simulink model "model"  (R2016a)
(part 5 of 5)

  _CN_100861711_400000_CN_90547679_400000/RConn1 -- T_100861711_400000_Keadby_400kV_Substation/LConn1 -- _CN_100861711_400000_CN_257311344_400000/LConn1 -- _CN_100861711_400000_CN_160279525_400000/LConn1 -- _CN_100861711_400000_CN_204918278_400000/LConn1 -- _CN_100861711_400000_CN_205132633_400000/LConn1 -- _CN_100861711_400000_CN_33917128_400000/LConn1 -- _CN_100861711_400000_CN_58736682_400000/LConn1 -- _CN_100861711_400000_CN_324880597_400000/LConn1 -- _CN_100861711_400000_CN_159736514_400000/LConn1 -- _CN_100861711_400000_CN_34383063_400000/LConn1
  _CN_100861711_400000_CN_90547679_400000/RConn2 -- T_100861711_400000_Keadby_400kV_Substation/LConn2 -- _CN_100861711_400000_CN_257311344_400000/LConn2 -- _CN_100861711_400000_CN_160279525_400000/LConn2 -- _CN_100861711_400000_CN_204918278_400000/LConn2 -- _CN_100861711_400000_CN_205132633_400000/LConn2 -- _CN_100861711_400000_CN_33917128_400000/LConn2 -- _CN_100861711_400000_CN_58736682_400000/LConn2 -- _CN_100861711_400000_CN_324880597_400000/LConn2 -- _CN_100861711_400000_CN_159736514_400000/LConn2 -- _CN_100861711_400000_CN_34383063_400000/LConn2
  _CN_100861711_400000_CN_90547679_400000/RConn3 -- T_100861711_400000_Keadby_400kV_Substation/LConn3 -- _CN_100861711_400000_CN_257311344_400000/LConn3 -- _CN_100861711_400000_CN_160279525_400000/LConn3 -- _CN_100861711_400000_CN_204918278_400000/LConn3 -- _CN_100861711_400000_CN_205132633_400000/LConn3 -- _CN_100861711_400000_CN_33917128_400000/LConn3 -- _CN_100861711_400000_CN_58736682_400000/LConn3 -- _CN_100861711_400000_CN_324880597_400000/LConn3 -- bus109/LConn1 -- _CN_100861711_400000_CN_159736514_400000/LConn3 -- _CN_100861711_400000_CN_34383063_400000/LConn3
  T_159736514_400000;275000_Brinsworth_Switching_Station/LConn1 -- _CN_100861711_400000_CN_159736514_400000/RConn1
  T_159736514_400000;275000_Brinsworth_Switching_Station/LConn2 -- _CN_100861711_400000_CN_159736514_400000/RConn2
  _CN_100861711_400000_CN_159736514_400000/RConn3 -- T_159736514_400000;275000_Brinsworth_Switching_Station/LConn3 -- bus110/LConn1
  _CN_100861711_400000_CN_34383063_400000/RConn1 -- G_34383063_Drax_power_station/RConn1 -- _CN_160580052_400000_CN_34383063_400000/LConn1 -- _CN_25629803_400000_CN_34383063_400000/LConn1 -- _CN_313495269_400000_CN_34383063_400000/LConn1
  _CN_100861711_400000_CN_34383063_400000/RConn2 -- G_34383063_Drax_power_station/RConn2 -- _CN_160580052_400000_CN_34383063_400000/LConn2 -- _CN_25629803_400000_CN_34383063_400000/LConn2 -- _CN_313495269_400000_CN_34383063_400000/LConn2
  _CN_100861711_400000_CN_34383063_400000/RConn3 -- G_34383063_Drax_power_station/RConn3 -- _CN_160580052_400000_CN_34383063_400000/LConn3 -- bus111/LConn1 -- _CN_25629803_400000_CN_34383063_400000/LConn3 -- _CN_313495269_400000_CN_34383063_400000/LConn3
  T_257311344_400000;132000_/LConn1 -- _CN_100861711_400000_CN_257311344_400000/RConn1
  T_257311344_400000;132000_/LConn2 -- _CN_100861711_400000_CN_257311344_400000/RConn2
  _CN_100861711_400000_CN_257311344_400000/RConn3 -- T_257311344_400000;132000_/LConn3 -- bus112/LConn1
  T_160279525_400000;132000_Grimsby_West_Substation/LConn1 -- _CN_100861711_400000_CN_160279525_400000/RConn1
  T_160279525_400000;132000_Grimsby_West_Substation/LConn2 -- _CN_100861711_400000_CN_160279525_400000/RConn2
  _CN_100861711_400000_CN_160279525_400000/RConn3 -- T_160279525_400000;132000_Grimsby_West_Substation/LConn3 -- bus113/LConn1
  _CN_100861711_400000_CN_204918278_400000/RConn1 -- G_204918278_South_Humber_Bank_Power_Station/RConn1 -- _CN_313180501_400000_CN_204918278_400000/LConn1
  _CN_100861711_400000_CN_204918278_400000/RConn2 -- G_204918278_South_Humber_Bank_Power_Station/RConn2 -- _CN_313180501_400000_CN_204918278_400000/LConn2
  _CN_100861711_400000_CN_204918278_400000/RConn3 -- G_204918278_South_Humber_Bank_Power_Station/RConn3 -- _CN_313180501_400000_CN_204918278_400000/LConn3 -- bus114/LConn1
  T_205132633_400000_/LConn1 -- _CN_100861711_400000_CN_205132633_400000/RConn1
  T_205132633_400000_/LConn2 -- _CN_100861711_400000_CN_205132633_400000/RConn2
  _CN_100861711_400000_CN_205132633_400000/RConn3 -- T_205132633_400000_/LConn3 -- bus115/LConn1
  _CN_100861711_400000_CN_33917128_400000/RConn1 -- T_33917128_400000;275000;132000_Creyke_Beck_Substation/LConn1 -- _CN_25629803_400000_CN_33917128_400000/LConn1
  _CN_100861711_400000_CN_33917128_400000/RConn2 -- T_33917128_400000;275000;132000_Creyke_Beck_Substation/LConn2 -- _CN_25629803_400000_CN_33917128_400000/LConn2
  _CN_100861711_400000_CN_33917128_400000/RConn3 -- T_33917128_400000;275000;132000_Creyke_Beck_Substation/LConn3 -- _CN_25629803_400000_CN_33917128_400000/LConn3 -- bus116/LConn1
  G_58736682_Keadby_Power_Station/RConn1 -- _CN_100861711_400000_CN_58736682_400000/RConn1
  G_58736682_Keadby_Power_Station/RConn2 -- _CN_100861711_400000_CN_58736682_400000/RConn2
  _CN_100861711_400000_CN_58736682_400000/RConn3 -- G_58736682_Keadby_Power_Station/RConn3 -- bus117/LConn1
  _CN_100861711_400000_CN_324880597_400000/RConn1 -- G_324880597_West_Burton_A_Coal_Power_Station/RConn1 -- _CN_190511290_400000_CN_324880597_400000/LConn1 -- _CN_314338799_400000_CN_324880597_400000/LConn1
  _CN_100861711_400000_CN_324880597_400000/RConn2 -- G_324880597_West_Burton_A_Coal_Power_Station/RConn2 -- _CN_190511290_400000_CN_324880597_400000/LConn2 -- _CN_314338799_400000_CN_324880597_400000/LConn2
  _CN_100861711_400000_CN_324880597_400000/RConn3 -- G_324880597_West_Burton_A_Coal_Power_Station/RConn3 -- _CN_190511290_400000_CN_324880597_400000/LConn3 -- _CN_314338799_400000_CN_324880597_400000/LConn3 -- bus118/LConn1
  T_264650878__/LConn1 -- _CN_264650844_400000_CN_264650878_400000/RConn1
  T_264650878__/LConn2 -- _CN_264650844_400000_CN_264650878_400000/RConn2
  _CN_264650844_400000_CN_264650878_400000/RConn3 -- T_264650878__/LConn3 -- bus119/LConn1
  _CN_143783006_400000_CN_150780483_400000/LConn1 -- T_143783006_400000_/LConn1 -- _CN_143783006_400000_CN_10270618_400000/RConn1
  _CN_143783006_400000_CN_150780483_400000/LConn2 -- T_143783006_400000_/LConn2 -- _CN_143783006_400000_CN_10270618_400000/RConn2
  _CN_143783006_400000_CN_150780483_400000/LConn3 -- T_143783006_400000_/LConn3 -- _CN_143783006_400000_CN_10270618_400000/RConn3 -- bus120/LConn1
  G_150780483_Medway_Power_Station/RConn1 -- _CN_143783006_400000_CN_150780483_400000/RConn1
  G_150780483_Medway_Power_Station/RConn2 -- _CN_143783006_400000_CN_150780483_400000/RConn2
  _CN_143783006_400000_CN_150780483_400000/RConn3 -- G_150780483_Medway_Power_Station/RConn3 -- bus121/LConn1
  Dungeness_Ninfield_CN_28691559_400000_CN_88540693_400000/RConn1 -- T_28691559_400000;132000_Ninfield_Substation/LConn1 -- National_Grid_Bolney_Ninfield_CN_28691559_400000_CN_91082448_400000/LConn1
  Dungeness_Ninfield_CN_28691559_400000_CN_88540693_400000/RConn2 -- T_28691559_400000;132000_Ninfield_Substation/LConn2 -- National_Grid_Bolney_Ninfield_CN_28691559_400000_CN_91082448_400000/LConn2
  Dungeness_Ninfield_CN_28691559_400000_CN_88540693_400000/RConn3 -- T_28691559_400000;132000_Ninfield_Substation/LConn3 -- National_Grid_Bolney_Ninfield_CN_28691559_400000_CN_91082448_400000/LConn3 -- bus122/LConn1
  National_Grid_Bolney_Ninfield_CN_28691559_400000_CN_91082448_400000/RConn1 -- T_91082448_400000;132000_Bolney_Substation/LConn1 -- Bolney_Lovedean_CN_91082448_400000_CN_20851038_400000/RConn1
  National_Grid_Bolney_Ninfield_CN_28691559_400000_CN_91082448_400000/RConn2 -- T_91082448_400000;132000_Bolney_Substation/LConn2 -- Bolney_Lovedean_CN_91082448_400000_CN_20851038_400000/RConn2
  National_Grid_Bolney_Ninfield_CN_28691559_400000_CN_91082448_400000/RConn3 -- T_91082448_400000;132000_Bolney_Substation/LConn3 -- Bolney_Lovedean_CN_91082448_400000_CN_20851038_400000/RConn3 -- bus123/LConn1
  G_402566315_Cottam_Power_Station/RConn1 -- _CN_314338790_400000_CN_402566315_400000/RConn1
  G_402566315_Cottam_Power_Station/RConn2 -- _CN_314338790_400000_CN_402566315_400000/RConn2
  _CN_314338790_400000_CN_402566315_400000/RConn3 -- G_402566315_Cottam_Power_Station/RConn3 -- bus124/LConn1
  _CN_25629803_400000_CN_90125443_400000/LConn1 -- T_25629803_400000_Thornton_Substation/LConn1 -- _CN_25629803_400000_CN_33917128_400000/RConn1 -- _CN_25629803_400000_CN_209404646_400000/LConn1 -- _CN_25629803_400000_CN_34383063_400000/RConn1
  _CN_25629803_400000_CN_90125443_400000/LConn2 -- T_25629803_400000_Thornton_Substation/LConn2 -- _CN_25629803_400000_CN_33917128_400000/RConn2 -- _CN_25629803_400000_CN_209404646_400000/LConn2 -- _CN_25629803_400000_CN_34383063_400000/RConn2
  _CN_25629803_400000_CN_90125443_400000/LConn3 -- T_25629803_400000_Thornton_Substation/LConn3 -- _CN_25629803_400000_CN_33917128_400000/RConn3 -- _CN_25629803_400000_CN_209404646_400000/LConn3 -- bus125/LConn1 -- _CN_25629803_400000_CN_34383063_400000/RConn3
  _CN_25629803_400000_CN_90125443_400000/RConn1 -- T_90125443_400000_/LConn1 -- _CN_90125443_400000_CN_43472283_400000/LConn1
  _CN_25629803_400000_CN_90125443_400000/RConn2 -- T_90125443_400000_/LConn2 -- _CN_90125443_400000_CN_43472283_400000/LConn2
  _CN_25629803_400000_CN_90125443_400000/RConn3 -- T_90125443_400000_/LConn3 -- _CN_90125443_400000_CN_43472283_400000/LConn3 -- bus126/LConn1
  _CN_25629803_400000_CN_209404646_400000/RConn1 -- T_209404646__/LConn1 -- _CN_142397822_400000_CN_209404646_400000/LConn1
  _CN_25629803_400000_CN_209404646_400000/RConn2 -- T_209404646__/LConn2 -- _CN_142397822_400000_CN_209404646_400000/LConn2
  _CN_25629803_400000_CN_209404646_400000/RConn3 -- T_209404646__/LConn3 -- _CN_142397822_400000_CN_209404646_400000/LConn3 -- bus127/LConn1
  _CN_45357172_400000_CN_94004582_400000/RConn1 -- T_45357172_400000;132000_Hutton_Substation/LConn1 -- _CN_45357172_400000_CN_81048391_400000/RConn1 -- _CN_45357172_400000_CN_88799419_400000/RConn1
  _CN_45357172_400000_CN_94004582_400000/RConn2 -- T_45357172_400000;132000_Hutton_Substation/LConn2 -- _CN_45357172_400000_CN_81048391_400000/RConn2 -- _CN_45357172_400000_CN_88799419_400000/RConn2
  _CN_45357172_400000_CN_94004582_400000/RConn3 -- T_45357172_400000;132000_Hutton_Substation/LConn3 -- _CN_45357172_400000_CN_81048391_400000/RConn3 -- _CN_45357172_400000_CN_88799419_400000/RConn3 -- bus128/LConn1
  _CN_88389243_400000_CN_20851038_400000/RConn1 -- T_88389243_400000;132000_Fleet_Substation/LConn1 -- _CN_88389243_400000_CN_32796576_400000/LConn1
  _CN_88389243_400000_CN_20851038_400000/RConn2 -- T_88389243_400000;132000_Fleet_Substation/LConn2 -- _CN_88389243_400000_CN_32796576_400000/LConn2
  _CN_88389243_400000_CN_20851038_400000/RConn3 -- T_88389243_400000;132000_Fleet_Substation/LConn3 -- _CN_88389243_400000_CN_32796576_400000/LConn3 -- bus129/LConn1
  _CN_88389243_400000_CN_32796576_400000/RConn1 -- T_32796576_400000;132000_Bramley_Substation/LConn1 -- National_Grid_Bramley_Melksham_CN_103915328_400000_CN_32796576_400000/RConn1 -- National_Grid_Didcot_Bramley_CN_32796576_400000_CN_160173034_400000/LConn1 -- National_Grid_Bramley_West_Weybridge_CN_144135298_400000_CN_32796576_400000/LConn1
  _CN_88389243_400000_CN_32796576_400000/RConn2 -- T_32796576_400000;132000_Bramley_Substation/LConn2 -- National_Grid_Bramley_Melksham_CN_103915328_400000_CN_32796576_400000/RConn2 -- National_Grid_Didcot_Bramley_CN_32796576_400000_CN_160173034_400000/LConn2 -- National_Grid_Bramley_West_Weybridge_CN_144135298_400000_CN_32796576_400000/LConn2
  _CN_88389243_400000_CN_32796576_400000/RConn3 -- T_32796576_400000;132000_Bramley_Substation/LConn3 -- National_Grid_Bramley_Melksham_CN_103915328_400000_CN_32796576_400000/RConn3 -- National_Grid_Didcot_Bramley_CN_32796576_400000_CN_160173034_400000/LConn3 -- bus130/LConn1 -- National_Grid_Bramley_West_Weybridge_CN_144135298_400000_CN_32796576_400000/LConn3
  _CN_92737152_400000_CN_293585872_400000/RConn1 -- T_293585872__/LConn1 -- _CN_293585871_400000_CN_293585872_400000/RConn1
  _CN_92737152_400000_CN_293585872_400000/RConn2 -- T_293585872__/LConn2 -- _CN_293585871_400000_CN_293585872_400000/RConn2
  _CN_92737152_400000_CN_293585872_400000/RConn3 -- T_293585872__/LConn3 -- _CN_293585871_400000_CN_293585872_400000/RConn3 -- bus131/LConn1
  T_264650881__/LConn1 -- National_Grid_Bramford_?_CN_264650881_400000_CN_32227788_400000/LConn1
  T_264650881__/LConn2 -- National_Grid_Bramford_?_CN_264650881_400000_CN_32227788_400000/LConn2
  National_Grid_Bramford_?_CN_264650881_400000_CN_32227788_400000/LConn3 -- T_264650881__/LConn3 -- bus132/LConn1
  National_Grid_Bramford_?_CN_264650881_400000_CN_32227788_400000/RConn1 -- T_32227788_400000_Norwich_Main_Substation/LConn1 -- _CN_38528291_400000_CN_32227788_400000/RConn1
  National_Grid_Bramford_?_CN_264650881_400000_CN_32227788_400000/RConn2 -- T_32227788_400000_Norwich_Main_Substation/LConn2 -- _CN_38528291_400000_CN_32227788_400000/RConn2
  National_Grid_Bramford_?_CN_264650881_400000_CN_32227788_400000/RConn3 -- T_32227788_400000_Norwich_Main_Substation/LConn3 -- _CN_38528291_400000_CN_32227788_400000/RConn3 -- bus133/LConn1
  T_144135298_400000;275000_West_Weybridge_Substation/LConn1 -- National_Grid_Bramley_West_Weybridge_CN_144135298_400000_CN_32796576_400000/RConn1
  T_144135298_400000;275000_West_Weybridge_Substation/LConn2 -- National_Grid_Bramley_West_Weybridge_CN_144135298_400000_CN_32796576_400000/RConn2
  National_Grid_Bramley_West_Weybridge_CN_144135298_400000_CN_32796576_400000/RConn3 -- T_144135298_400000;275000_West_Weybridge_Substation/LConn3 -- bus134/LConn1
  _CN_90125443_400000_CN_43472283_400000/RConn1 -- T_43472283_400000;132000_Norton_Sub_Station/LConn1 -- _CN_43472283_400000_CN_109730296_400000/LConn1 -- _CN_220798107_400000_CN_43472283_400000/LConn1 -- _CN_200511209_400000_CN_43472283_400000/LConn1
  _CN_90125443_400000_CN_43472283_400000/RConn2 -- T_43472283_400000;132000_Norton_Sub_Station/LConn2 -- _CN_43472283_400000_CN_109730296_400000/LConn2 -- _CN_220798107_400000_CN_43472283_400000/LConn2 -- _CN_200511209_400000_CN_43472283_400000/LConn2
  _CN_90125443_400000_CN_43472283_400000/RConn3 -- T_43472283_400000;132000_Norton_Sub_Station/LConn3 -- _CN_43472283_400000_CN_109730296_400000/LConn3 -- bus135/LConn1 -- _CN_220798107_400000_CN_43472283_400000/LConn3 -- _CN_200511209_400000_CN_43472283_400000/LConn3
  _CN_94583940_400000_CN_23167368_400000/LConn1 -- T_94583940__/LConn1 -- _CN_94583940_400000_CN_195575988_400000/LConn1
  _CN_94583940_400000_CN_23167368_400000/LConn2 -- T_94583940__/LConn2 -- _CN_94583940_400000_CN_195575988_400000/LConn2
  _CN_94583940_400000_CN_23167368_400000/LConn3 -- T_94583940__/LConn3 -- _CN_94583940_400000_CN_195575988_400000/LConn3 -- bus136/LConn1
  _CN_94583940_400000_CN_23167368_400000/RConn1 -- T_23167368_400000_Connahs_Quay_Substation/LConn1 -- _CN_98899051_400000_CN_23167368_400000/LConn1 -- _CN_95338682_400000_CN_23167368_400000/LConn1 -- _CN_23164132_400000_CN_23167368_400000/LConn1
  _CN_94583940_400000_CN_23167368_400000/RConn2 -- T_23167368_400000_Connahs_Quay_Substation/LConn2 -- _CN_98899051_400000_CN_23167368_400000/LConn2 -- _CN_95338682_400000_CN_23167368_400000/LConn2 -- _CN_23164132_400000_CN_23167368_400000/LConn2
  _CN_94583940_400000_CN_23167368_400000/RConn3 -- T_23167368_400000_Connahs_Quay_Substation/LConn3 -- _CN_98899051_400000_CN_23167368_400000/LConn3 -- bus137/LConn1 -- _CN_95338682_400000_CN_23167368_400000/LConn3 -- _CN_23164132_400000_CN_23167368_400000/LConn3
  _CN_94583940_400000_CN_195575988_400000/RConn1 -- G_195575988_Deeside_Power_Station/RConn1 -- _CN_23167419_400000_CN_195575988_400000/LConn1
  _CN_94583940_400000_CN_195575988_400000/RConn2 -- G_195575988_Deeside_Power_Station/RConn2 -- _CN_23167419_400000_CN_195575988_400000/LConn2
  _CN_94583940_400000_CN_195575988_400000/RConn3 -- G_195575988_Deeside_Power_Station/RConn3 -- _CN_23167419_400000_CN_195575988_400000/LConn3 -- bus138/LConn1
  National_Grid_Chilling_Fawley_CN_23309078_400000_CN_5728891_400000/RConn1 -- T_23309078_400000_Chilling_Substation/LConn1 -- National_Grid_Chilling_Fawley_CN_23309078_400000_CN_23300984_400000/LConn1
  National_Grid_Chilling_Fawley_CN_23309078_400000_CN_5728891_400000/RConn2 -- T_23309078_400000_Chilling_Substation/LConn2 -- National_Grid_Chilling_Fawley_CN_23309078_400000_CN_23300984_400000/LConn2
  National_Grid_Chilling_Fawley_CN_23309078_400000_CN_5728891_400000/RConn3 -- T_23309078_400000_Chilling_Substation/LConn3 -- National_Grid_Chilling_Fawley_CN_23309078_400000_CN_23300984_400000/LConn3 -- bus139/LConn1
  National_Grid_Chilling_Fawley_CN_23309078_400000_CN_23300984_400000/RConn1 -- T_23300984_400000_Chilling_Substation/LConn1 -- _CN_23300984_400000_CN_20851038_400000/RConn1 -- _CN_23300984_400000_CN_4715504_400000/LConn1
  National_Grid_Chilling_Fawley_CN_23309078_400000_CN_23300984_400000/RConn2 -- T_23300984_400000_Chilling_Substation/LConn2 -- _CN_23300984_400000_CN_20851038_400000/RConn2 -- _CN_23300984_400000_CN_4715504_400000/LConn2
  National_Grid_Chilling_Fawley_CN_23309078_400000_CN_23300984_400000/RConn3 -- T_23300984_400000_Chilling_Substation/LConn3 -- _CN_23300984_400000_CN_20851038_400000/RConn3 -- _CN_23300984_400000_CN_4715504_400000/LConn3 -- bus140/LConn1
  National_Grid_Daines_Macclesfield_CN_142738881_400000_CN_92529432_400000/RConn1 -- T_142738881__/LConn1 -- National_Grid_Daines_Macclesfield_(underground)_CN_142738881_400000_CN_142738882_400000/LConn1
  National_Grid_Daines_Macclesfield_CN_142738881_400000_CN_92529432_400000/RConn2 -- T_142738881__/LConn2 -- National_Grid_Daines_Macclesfield_(underground)_CN_142738881_400000_CN_142738882_400000/LConn2
  National_Grid_Daines_Macclesfield_CN_142738881_400000_CN_92529432_400000/RConn3 -- T_142738881__/LConn3 -- National_Grid_Daines_Macclesfield_(underground)_CN_142738881_400000_CN_142738882_400000/LConn3 -- bus141/LConn1
  National_Grid_Daines_Macclesfield_(underground)_CN_142738881_400000_CN_142738882_400000/RConn1 -- T_142738882__/LConn1 -- National_Grid_Macclesfield_?_CN_92419253_400000_CN_142738882_400000/LConn1
  National_Grid_Daines_Macclesfield_(underground)_CN_142738881_400000_CN_142738882_400000/RConn2 -- T_142738882__/LConn2 -- National_Grid_Macclesfield_?_CN_92419253_400000_CN_142738882_400000/LConn2
  National_Grid_Daines_Macclesfield_(underground)_CN_142738881_400000_CN_142738882_400000/RConn3 -- T_142738882__/LConn3 -- National_Grid_Macclesfield_?_CN_92419253_400000_CN_142738882_400000/LConn3 -- bus142/LConn1
  _CN_291629706_400000_CN_147672722_400000/RConn1 -- T_147672722_400000_/LConn1 -- _CN_147672722_400000_CN_95159241_400000/LConn1
  _CN_291629706_400000_CN_147672722_400000/RConn2 -- T_147672722_400000_/LConn2 -- _CN_147672722_400000_CN_95159241_400000/LConn2
  _CN_291629706_400000_CN_147672722_400000/RConn3 -- T_147672722_400000_/LConn3 -- _CN_147672722_400000_CN_95159241_400000/LConn3 -- bus143/LConn1
  T_100009331_400000;132000_Alverdiscott_Substation/LConn1 -- _CN_143791249_400000_CN_100009331_400000/RConn1
  T_100009331_400000;132000_Alverdiscott_Substation/LConn2 -- _CN_143791249_400000_CN_100009331_400000/RConn2
  _CN_143791249_400000_CN_100009331_400000/RConn3 -- T_100009331_400000;132000_Alverdiscott_Substation/LConn3 -- bus144/LConn1
  _CN_143791249_400000_CN_34656007_400000/RConn1 -- T_34656007_400000;132000_Landulph_Substation/LConn1 -- _CN_34656007_400000_CN_26938722_400000/LConn1
  _CN_143791249_400000_CN_34656007_400000/RConn2 -- T_34656007_400000;132000_Landulph_Substation/LConn2 -- _CN_34656007_400000_CN_26938722_400000/LConn2
  _CN_143791249_400000_CN_34656007_400000/RConn3 -- T_34656007_400000;132000_Landulph_Substation/LConn3 -- _CN_34656007_400000_CN_26938722_400000/LConn3 -- bus145/LConn1
  G_143791247_Indian_Queens_Power_Station/RConn1 -- _CN_143791249_400000_CN_143791247_400000/RConn1
  G_143791247_Indian_Queens_Power_Station/RConn2 -- _CN_143791249_400000_CN_143791247_400000/RConn2
  _CN_143791249_400000_CN_143791247_400000/RConn3 -- G_143791247_Indian_Queens_Power_Station/RConn3 -- bus146/LConn1
  T_95159241_400000;275000_/LConn1 -- _CN_147672722_400000_CN_95159241_400000/RConn1
  T_95159241_400000;275000_/LConn2 -- _CN_147672722_400000_CN_95159241_400000/RConn2
  _CN_147672722_400000_CN_95159241_400000/RConn3 -- T_95159241_400000;275000_/LConn3 -- bus147/LConn1
  T_89427607_400000_Transformer_House/LConn1 -- National_Grid_Wylfa_Pentir_CN_89427607_400000_CN_98899051_400000/LConn1
  T_89427607_400000_Transformer_House/LConn2 -- National_Grid_Wylfa_Pentir_CN_89427607_400000_CN_98899051_400000/LConn2
  National_Grid_Wylfa_Pentir_CN_89427607_400000_CN_98899051_400000/LConn3 -- T_89427607_400000_Transformer_House/LConn3 -- bus148/LConn1
  National_Grid_Wylfa_Pentir_CN_89427607_400000_CN_98899051_400000/RConn1 -- T_98899051_400000;132000_Pentir_Substation/LConn1 -- _CN_98899051_400000_CN_23167368_400000/RConn1 -- National_Grid_Pentir_Trawsfynydd_CN_98899051_400000_CN_142845284_400000/LConn1 -- National_Grid_Pentir_Trawsfynydd_CN_98899051_400000_CN_142843255_400000/LConn1
  National_Grid_Wylfa_Pentir_CN_89427607_400000_CN_98899051_400000/RConn2 -- T_98899051_400000;132000_Pentir_Substation/LConn2 -- _CN_98899051_400000_CN_23167368_400000/RConn2 -- National_Grid_Pentir_Trawsfynydd_CN_98899051_400000_CN_142845284_400000/LConn2 -- National_Grid_Pentir_Trawsfynydd_CN_98899051_400000_CN_142843255_400000/LConn2
  National_Grid_Wylfa_Pentir_CN_89427607_400000_CN_98899051_400000/RConn3 -- T_98899051_400000;132000_Pentir_Substation/LConn3 -- _CN_98899051_400000_CN_23167368_400000/RConn3 -- bus149/LConn1 -- National_Grid_Pentir_Trawsfynydd_CN_98899051_400000_CN_142845284_400000/LConn3 -- National_Grid_Pentir_Trawsfynydd_CN_98899051_400000_CN_142843255_400000/LConn3
  _CN_220798107_400000_CN_43472283_400000/RConn1 -- T_220798107_400000;132000_Spennymoor_Substation/LConn1 -- _CN_220798107_400000_CN_91955171_400000/RConn1
  _CN_220798107_400000_CN_43472283_400000/RConn2 -- T_220798107_400000;132000_Spennymoor_Substation/LConn2 -- _CN_220798107_400000_CN_91955171_400000/RConn2
  _CN_220798107_400000_CN_43472283_400000/RConn3 -- T_220798107_400000;132000_Spennymoor_Substation/LConn3 -- _CN_220798107_400000_CN_91955171_400000/RConn3 -- bus150/LConn1
  _CN_97551518_400000_CN_91104903_400000/RConn1 -- G_91104903_Torness_Nuclear_Power_Station/RConn1 -- _CN_97551523_400000_CN_91104903_400000/RConn1
  _CN_97551518_400000_CN_91104903_400000/RConn2 -- G_91104903_Torness_Nuclear_Power_Station/RConn2 -- _CN_97551523_400000_CN_91104903_400000/RConn2
  _CN_97551518_400000_CN_91104903_400000/RConn3 -- G_91104903_Torness_Nuclear_Power_Station/RConn3 -- _CN_97551523_400000_CN_91104903_400000/RConn3 -- bus151/LConn1
  _CN_87204522_400000_CN_35287066_400000/RConn1 -- T_87204522_400000;275000;132000_Drakelow_Substation/LConn1 -- _CN_87204522_400000_CN_87207123_400000/LConn1 -- _CN_87204522_400000_CN_142741752_400000/LConn1 -- _CN_87204522_400000_CN_165506012_400000/LConn1 -- _CN_87204522_400000_CN_92458761_400000/LConn1 -- _CN_87204522_400000_CN_221490974_400000/LConn1 -- _CN_87204522_400000_CN_277887478_400000/LConn1 -- _CN_87204522_400000_CN_49499923_400000/LConn1 -- _CN_87204522_400000_CN_167621580_400000/LConn1
  _CN_87204522_400000_CN_35287066_400000/RConn2 -- T_87204522_400000;275000;132000_Drakelow_Substation/LConn2 -- _CN_87204522_400000_CN_87207123_400000/LConn2 -- _CN_87204522_400000_CN_142741752_400000/LConn2 -- _CN_87204522_400000_CN_165506012_400000/LConn2 -- _CN_87204522_400000_CN_92458761_400000/LConn2 -- _CN_87204522_400000_CN_221490974_400000/LConn2 -- _CN_87204522_400000_CN_277887478_400000/LConn2 -- _CN_87204522_400000_CN_49499923_400000/LConn2 -- _CN_87204522_400000_CN_167621580_400000/LConn2
  _CN_87204522_400000_CN_35287066_400000/RConn3 -- T_87204522_400000;275000;132000_Drakelow_Substation/LConn3 -- _CN_87204522_400000_CN_87207123_400000/LConn3 -- _CN_87204522_400000_CN_142741752_400000/LConn3 -- _CN_87204522_400000_CN_165506012_400000/LConn3 -- _CN_87204522_400000_CN_92458761_400000/LConn3 -- bus152/LConn1 -- _CN_87204522_400000_CN_221490974_400000/LConn3 -- _CN_87204522_400000_CN_277887478_400000/LConn3 -- _CN_87204522_400000_CN_49499923_400000/LConn3 -- _CN_87204522_400000_CN_167621580_400000/LConn3
  _CN_87204522_400000_CN_221490974_400000/RConn1 -- T_221490974__/LConn1 -- _CN_221490974_400000_CN_49499923_400000/LConn1
  _CN_87204522_400000_CN_221490974_400000/RConn2 -- T_221490974__/LConn2 -- _CN_221490974_400000_CN_49499923_400000/LConn2
  _CN_87204522_400000_CN_221490974_400000/RConn3 -- T_221490974__/LConn3 -- _CN_221490974_400000_CN_49499923_400000/LConn3 -- bus153/LConn1
  _CN_87204522_400000_CN_277887478_400000/RConn1 -- T_277887478_400000_Willington_Substation/LConn1 -- _CN_277887478_400000_CN_35287066_400000/RConn1
  _CN_87204522_400000_CN_277887478_400000/RConn2 -- T_277887478_400000_Willington_Substation/LConn2 -- _CN_277887478_400000_CN_35287066_400000/RConn2
  _CN_87204522_400000_CN_277887478_400000/RConn3 -- T_277887478_400000_Willington_Substation/LConn3 -- _CN_277887478_400000_CN_35287066_400000/RConn3 -- bus154/LConn1
  _CN_87204522_400000_CN_49499923_400000/RConn1 -- T_49499923_400000;275000_Hams_Hall_Substation/LConn1 -- _CN_221490974_400000_CN_49499923_400000/RConn1 -- _CN_49499923_400000_CN_96107758_400000/LConn1
  _CN_87204522_400000_CN_49499923_400000/RConn2 -- T_49499923_400000;275000_Hams_Hall_Substation/LConn2 -- _CN_221490974_400000_CN_49499923_400000/RConn2 -- _CN_49499923_400000_CN_96107758_400000/LConn2
  _CN_87204522_400000_CN_49499923_400000/RConn3 -- T_49499923_400000;275000_Hams_Hall_Substation/LConn3 -- _CN_221490974_400000_CN_49499923_400000/RConn3 -- _CN_49499923_400000_CN_96107758_400000/LConn3 -- bus155/LConn1
  T_167621580_400000;275000;132000_/LConn1 -- _CN_87204522_400000_CN_167621580_400000/RConn1
  T_167621580_400000;275000;132000_/LConn2 -- _CN_87204522_400000_CN_167621580_400000/RConn2
  _CN_87204522_400000_CN_167621580_400000/RConn3 -- T_167621580_400000;275000;132000_/LConn3 -- bus156/LConn1
  _CN_87204522_400000_CN_87207123_400000/RConn1 -- T_87207123_400000;132000_Cellarhead_Substation/LConn1 -- National_Grid_Macclesfield_?_CN_92419253_400000_CN_87207123_400000/LConn1
  _CN_87204522_400000_CN_87207123_400000/RConn2 -- T_87207123_400000;132000_Cellarhead_Substation/LConn2 -- National_Grid_Macclesfield_?_CN_92419253_400000_CN_87207123_400000/LConn2
  _CN_87204522_400000_CN_87207123_400000/RConn3 -- T_87207123_400000;132000_Cellarhead_Substation/LConn3 -- National_Grid_Macclesfield_?_CN_92419253_400000_CN_87207123_400000/LConn3 -- bus157/LConn1
  T_142741752_400000_/LConn1 -- _CN_87204522_400000_CN_142741752_400000/RConn1
  T_142741752_400000_/LConn2 -- _CN_87204522_400000_CN_142741752_400000/RConn2
  _CN_87204522_400000_CN_142741752_400000/RConn3 -- T_142741752_400000_/LConn3 -- bus158/LConn1
  _CN_87204522_400000_CN_165506012_400000/RConn1 -- T_165506012_400000_/LConn1 -- _CN_92458761_400000_CN_165506012_400000/LConn1 -- _CN_95338682_400000_CN_165506012_400000/LConn1
  _CN_87204522_400000_CN_165506012_400000/RConn2 -- T_165506012_400000_/LConn2 -- _CN_92458761_400000_CN_165506012_400000/LConn2 -- _CN_95338682_400000_CN_165506012_400000/LConn2
  _CN_87204522_400000_CN_165506012_400000/RConn3 -- T_165506012_400000_/LConn3 -- _CN_92458761_400000_CN_165506012_400000/LConn3 -- bus159/LConn1 -- _CN_95338682_400000_CN_165506012_400000/LConn3
  _CN_87204522_400000_CN_92458761_400000/RConn1 -- T_92458761_400000;132000_Penn_Substation/LConn1 -- _CN_92458761_400000_CN_165506012_400000/RConn1 -- _CN_92458761_400000_CN_96107758_400000/LConn1
  _CN_87204522_400000_CN_92458761_400000/RConn2 -- T_92458761_400000;132000_Penn_Substation/LConn2 -- _CN_92458761_400000_CN_165506012_400000/RConn2 -- _CN_92458761_400000_CN_96107758_400000/LConn2
  _CN_87204522_400000_CN_92458761_400000/RConn3 -- T_92458761_400000;132000_Penn_Substation/LConn3 -- _CN_92458761_400000_CN_165506012_400000/RConn3 -- bus160/LConn1 -- _CN_92458761_400000_CN_96107758_400000/LConn3
  National_Grid_Macclesfield_?_CN_92419253_400000_CN_93878867_400000/RConn1 -- T_92419253_400000_Macclesfield_Substation/LConn1 -- National_Grid_Macclesfield_?_CN_92419253_400000_CN_142738882_400000/RConn1 -- National_Grid_Macclesfield_?_CN_92419253_400000_CN_87207123_400000/RConn1
  National_Grid_Macclesfield_?_CN_92419253_400000_CN_93878867_400000/RConn2 -- T_92419253_400000_Macclesfield_Substation/LConn2 -- National_Grid_Macclesfield_?_CN_92419253_400000_CN_142738882_400000/RConn2 -- National_Grid_Macclesfield_?_CN_92419253_400000_CN_87207123_400000/RConn2
  National_Grid_Macclesfield_?_CN_92419253_400000_CN_93878867_400000/RConn3 -- T_92419253_400000_Macclesfield_Substation/LConn3 -- National_Grid_Macclesfield_?_CN_92419253_400000_CN_142738882_400000/RConn3 -- National_Grid_Macclesfield_?_CN_92419253_400000_CN_87207123_400000/RConn3 -- bus161/LConn1
  _CN_95338682_400000_CN_165506012_400000/RConn1 -- T_95338682_400000;132000_Legacy_Substation/LConn1 -- _CN_95338682_400000_CN_127184694_400000/LConn1 -- _CN_95338682_400000_CN_89573357_400000/LConn1 -- _CN_95338682_400000_CN_23167368_400000/RConn1
  _CN_95338682_400000_CN_165506012_400000/RConn2 -- T_95338682_400000;132000_Legacy_Substation/LConn2 -- _CN_95338682_400000_CN_127184694_400000/LConn2 -- _CN_95338682_400000_CN_89573357_400000/LConn2 -- _CN_95338682_400000_CN_23167368_400000/RConn2
  _CN_95338682_400000_CN_165506012_400000/RConn3 -- T_95338682_400000;132000_Legacy_Substation/LConn3 -- _CN_95338682_400000_CN_127184694_400000/LConn3 -- _CN_95338682_400000_CN_89573357_400000/LConn3 -- _CN_95338682_400000_CN_23167368_400000/RConn3 -- bus162/LConn1
  T_127184694_400000;132000_/LConn1 -- _CN_95338682_400000_CN_127184694_400000/RConn1
  T_127184694_400000;132000_/LConn2 -- _CN_95338682_400000_CN_127184694_400000/RConn2
  _CN_95338682_400000_CN_127184694_400000/RConn3 -- T_127184694_400000;132000_/LConn3 -- bus163/LConn1
  T_89573357_400000;275000_Trawsfynydd_Substation/LConn1 -- _CN_95338682_400000_CN_89573357_400000/RConn1
  T_89573357_400000;275000_Trawsfynydd_Substation/LConn2 -- _CN_95338682_400000_CN_89573357_400000/RConn2
  _CN_95338682_400000_CN_89573357_400000/RConn3 -- T_89573357_400000;275000_Trawsfynydd_Substation/LConn3 -- bus164/LConn1
  T_193460855_400000_/LConn1 -- _CN_193460855_400000_CN_313495307_400000/LConn1
  T_193460855_400000_/LConn2 -- _CN_193460855_400000_CN_313495307_400000/LConn2
  _CN_193460855_400000_CN_313495307_400000/LConn3 -- T_193460855_400000_/LConn3 -- bus165/LConn1
  _CN_193460855_400000_CN_313495307_400000/RConn1 -- G_313495307_Ferrybridge_C_Power_Station/RConn1 -- _CN_193617444_400000_CN_313495307_400000/RConn1 -- _CN_193460868_400000_CN_313495307_400000/LConn1 -- _CN_313495269_400000_CN_313495307_400000/LConn1
  _CN_193460855_400000_CN_313495307_400000/RConn2 -- G_313495307_Ferrybridge_C_Power_Station/RConn2 -- _CN_193617444_400000_CN_313495307_400000/RConn2 -- _CN_193460868_400000_CN_313495307_400000/LConn2 -- _CN_313495269_400000_CN_313495307_400000/LConn2
  _CN_193460855_400000_CN_313495307_400000/RConn3 -- G_313495307_Ferrybridge_C_Power_Station/RConn3 -- _CN_193617444_400000_CN_313495307_400000/RConn3 -- _CN_193460868_400000_CN_313495307_400000/LConn3 -- bus166/LConn1 -- _CN_313495269_400000_CN_313495307_400000/LConn3
  T_89038614_400000;132000_Eaton_Socon_substation/LConn1 -- _CN_24165071_400000_CN_89038614_400000/RConn1
  T_89038614_400000;132000_Eaton_Socon_substation/LConn2 -- _CN_24165071_400000_CN_89038614_400000/RConn2
  _CN_24165071_400000_CN_89038614_400000/RConn3 -- T_89038614_400000;132000_Eaton_Socon_substation/LConn3 -- bus167/LConn1
  G_154635235_Cottam_Power_Station/RConn1 -- _CN_24165071_400000_CN_154635235_400000/RConn1
  G_154635235_Cottam_Power_Station/RConn2 -- _CN_24165071_400000_CN_154635235_400000/RConn2
  _CN_24165071_400000_CN_154635235_400000/RConn3 -- G_154635235_Cottam_Power_Station/RConn3 -- bus168/LConn1
  T_4715504_400000;132000_Botley_Wood/LConn1 -- _CN_23300984_400000_CN_4715504_400000/RConn1
  T_4715504_400000;132000_Botley_Wood/LConn2 -- _CN_23300984_400000_CN_4715504_400000/RConn2
  _CN_23300984_400000_CN_4715504_400000/RConn3 -- T_4715504_400000;132000_Botley_Wood/LConn3 -- bus169/LConn1
  T_71118628_400000_/LConn1 -- _CN_71118628_400000_CN_35287066_400000/RConn1
  T_71118628_400000_/LConn2 -- _CN_71118628_400000_CN_35287066_400000/RConn2
  _CN_71118628_400000_CN_35287066_400000/RConn3 -- T_71118628_400000_/LConn3 -- bus170/LConn1
  _CN_264214748_400000_CN_103829261_400000/RConn1 -- T_103829261__/LConn1 -- National_Grid_Kingsnorth_Tilbury_CN_103829261_400000_CN_10270618_400000/RConn1 -- National_Grid_Kingsnorth_Tilbury_CN_103829261_400000_CN_88455233_400000/LConn1
  _CN_264214748_400000_CN_103829261_400000/RConn2 -- T_103829261__/LConn2 -- National_Grid_Kingsnorth_Tilbury_CN_103829261_400000_CN_10270618_400000/RConn2 -- National_Grid_Kingsnorth_Tilbury_CN_103829261_400000_CN_88455233_400000/LConn2
  _CN_264214748_400000_CN_103829261_400000/RConn3 -- T_103829261__/LConn3 -- National_Grid_Kingsnorth_Tilbury_CN_103829261_400000_CN_10270618_400000/RConn3 -- National_Grid_Kingsnorth_Tilbury_CN_103829261_400000_CN_88455233_400000/LConn3 -- bus171/LConn1
  National_Grid_Pentir_Trawsfynydd_(underground)_CN_137212453_400000_CN_89573358_400000/LConn1 -- T_137212453__/LConn1 -- National_Grid_Pentir_Trawsfynydd_(underground)_CN_137212453_400000_CN_142845284_400000/LConn1
  National_Grid_Pentir_Trawsfynydd_(underground)_CN_137212453_400000_CN_89573358_400000/LConn2 -- T_137212453__/LConn2 -- National_Grid_Pentir_Trawsfynydd_(underground)_CN_137212453_400000_CN_142845284_400000/LConn2
  National_Grid_Pentir_Trawsfynydd_(underground)_CN_137212453_400000_CN_89573358_400000/LConn3 -- T_137212453__/LConn3 -- National_Grid_Pentir_Trawsfynydd_(underground)_CN_137212453_400000_CN_142845284_400000/LConn3 -- bus172/LConn1
  T_89573358__/LConn1 -- National_Grid_Pentir_Trawsfynydd_(underground)_CN_137212453_400000_CN_89573358_400000/RConn1
  T_89573358__/LConn2 -- National_Grid_Pentir_Trawsfynydd_(underground)_CN_137212453_400000_CN_89573358_400000/RConn2
  National_Grid_Pentir_Trawsfynydd_(underground)_CN_137212453_400000_CN_89573358_400000/RConn3 -- T_89573358__/LConn3 -- bus173/LConn1
  National_Grid_Pentir_Trawsfynydd_(underground)_CN_137212453_400000_CN_142845284_400000/RConn1 -- T_142845284__/LConn1 -- National_Grid_Pentir_Trawsfynydd_CN_98899051_400000_CN_142845284_400000/RConn1
  National_Grid_Pentir_Trawsfynydd_(underground)_CN_137212453_400000_CN_142845284_400000/RConn2 -- T_142845284__/LConn2 -- National_Grid_Pentir_Trawsfynydd_CN_98899051_400000_CN_142845284_400000/RConn2
  National_Grid_Pentir_Trawsfynydd_(underground)_CN_137212453_400000_CN_142845284_400000/RConn3 -- T_142845284__/LConn3 -- National_Grid_Pentir_Trawsfynydd_CN_98899051_400000_CN_142845284_400000/RConn3 -- bus174/LConn1
  T_23232738_400000;275000_Iver_Substation/LConn1 -- _CN_23232738_400000_CN_41710456_400000/LConn1
  T_23232738_400000;275000_Iver_Substation/LConn2 -- _CN_23232738_400000_CN_41710456_400000/LConn2
  _CN_23232738_400000_CN_41710456_400000/LConn3 -- T_23232738_400000;275000_Iver_Substation/LConn3 -- bus175/LConn1
  _CN_23232738_400000_CN_41710456_400000/RConn1 -- T_41710456_400000;132000_Mop_End_Substation/LConn1 -- _CN_41710456_400000_CN_92340133_400000/LConn1
  _CN_23232738_400000_CN_41710456_400000/RConn2 -- T_41710456_400000;132000_Mop_End_Substation/LConn2 -- _CN_41710456_400000_CN_92340133_400000/LConn2
  _CN_23232738_400000_CN_41710456_400000/RConn3 -- T_41710456_400000;132000_Mop_End_Substation/LConn3 -- _CN_41710456_400000_CN_92340133_400000/LConn3 -- bus176/LConn1
  _CN_23164132_400000_CN_23167368_400000/RConn1 -- T_23164132_400000;275000;132000_/LConn1 -- National_Grid_Capenhurst_Frodsham_CN_23164132_400000_CN_23164256_400000/LConn1
  _CN_23164132_400000_CN_23167368_400000/RConn2 -- T_23164132_400000;275000;132000_/LConn2 -- National_Grid_Capenhurst_Frodsham_CN_23164132_400000_CN_23164256_400000/LConn2
  _CN_23164132_400000_CN_23167368_400000/RConn3 -- T_23164132_400000;275000;132000_/LConn3 -- National_Grid_Capenhurst_Frodsham_CN_23164132_400000_CN_23164256_400000/LConn3 -- bus177/LConn1
  T_23164256__/LConn1 -- National_Grid_Capenhurst_Frodsham_CN_23164132_400000_CN_23164256_400000/RConn1
  T_23164256__/LConn2 -- National_Grid_Capenhurst_Frodsham_CN_23164132_400000_CN_23164256_400000/RConn2
  National_Grid_Capenhurst_Frodsham_CN_23164132_400000_CN_23164256_400000/RConn3 -- T_23164256__/LConn3 -- bus178/LConn1
  _CN_313495269_400000_CN_313495305_400000/LConn1 -- T_313495269_400000_/LConn1 -- _CN_313495269_400000_CN_90547674_400000/RConn1 -- _CN_313495269_400000_CN_34383059_400000/RConn1 -- _CN_313495269_400000_CN_313495302_400000/LConn1 -- _CN_313495269_400000_CN_313495307_400000/RConn1 -- _CN_313495269_400000_CN_34383063_400000/RConn1
  _CN_313495269_400000_CN_313495305_400000/LConn2 -- T_313495269_400000_/LConn2 -- _CN_313495269_400000_CN_90547674_400000/RConn2 -- _CN_313495269_400000_CN_34383059_400000/RConn2 -- _CN_313495269_400000_CN_313495302_400000/LConn2 -- _CN_313495269_400000_CN_313495307_400000/RConn2 -- _CN_313495269_400000_CN_34383063_400000/RConn2
  _CN_313495269_400000_CN_313495305_400000/LConn3 -- T_313495269_400000_/LConn3 -- _CN_313495269_400000_CN_90547674_400000/RConn3 -- _CN_313495269_400000_CN_34383059_400000/RConn3 -- _CN_313495269_400000_CN_313495302_400000/LConn3 -- _CN_313495269_400000_CN_313495307_400000/RConn3 -- bus179/LConn1 -- _CN_313495269_400000_CN_34383063_400000/RConn3
  T_313495305__/LConn1 -- _CN_313495269_400000_CN_313495305_400000/RConn1
  T_313495305__/LConn2 -- _CN_313495269_400000_CN_313495305_400000/RConn2
  _CN_313495269_400000_CN_313495305_400000/RConn3 -- T_313495305__/LConn3 -- bus180/LConn1
  T_313495302__/LConn1 -- _CN_313495269_400000_CN_313495302_400000/RConn1
  T_313495302__/LConn2 -- _CN_313495269_400000_CN_313495302_400000/RConn2
  _CN_313495269_400000_CN_313495302_400000/RConn3 -- T_313495302__/LConn3 -- bus181/LConn1
  _CN_95279334_400000_CN_32117744_400000/RConn1 -- T_95279334_400000;132000_Minety/LConn1 -- _CN_95279334_400000_CN_92460913_400000/LConn1 -- _CN_95279334_400000_CN_96107758_400000/LConn1 -- _CN_95279334_400000_CN_103915328_400000/RConn1
  _CN_95279334_400000_CN_32117744_400000/RConn2 -- T_95279334_400000;132000_Minety/LConn2 -- _CN_95279334_400000_CN_92460913_400000/LConn2 -- _CN_95279334_400000_CN_96107758_400000/LConn2 -- _CN_95279334_400000_CN_103915328_400000/RConn2
  _CN_95279334_400000_CN_32117744_400000/RConn3 -- T_95279334_400000;132000_Minety/LConn3 -- _CN_95279334_400000_CN_92460913_400000/LConn3 -- _CN_95279334_400000_CN_96107758_400000/LConn3 -- _CN_95279334_400000_CN_103915328_400000/RConn3 -- bus182/LConn1
  _CN_95279334_400000_CN_92460913_400000/RConn1 -- T_92460913_400000_Walham_Sub_station/LConn1 -- _CN_92460913_400000_CN_92483460_400000/LConn1
  _CN_95279334_400000_CN_92460913_400000/RConn2 -- T_92460913_400000_Walham_Sub_station/LConn2 -- _CN_92460913_400000_CN_92483460_400000/LConn2
  _CN_95279334_400000_CN_92460913_400000/RConn3 -- T_92460913_400000_Walham_Sub_station/LConn3 -- _CN_92460913_400000_CN_92483460_400000/LConn3 -- bus183/LConn1
  _CN_95279334_400000_CN_96107758_400000/RConn1 -- T_96107758_400000;275000_Feckenham/LConn1 -- _CN_49499923_400000_CN_96107758_400000/RConn1 -- _CN_92458761_400000_CN_96107758_400000/RConn1
  _CN_95279334_400000_CN_96107758_400000/RConn2 -- T_96107758_400000;275000_Feckenham/LConn2 -- _CN_49499923_400000_CN_96107758_400000/RConn2 -- _CN_92458761_400000_CN_96107758_400000/RConn2
  _CN_95279334_400000_CN_96107758_400000/RConn3 -- T_96107758_400000;275000_Feckenham/LConn3 -- _CN_49499923_400000_CN_96107758_400000/RConn3 -- bus184/LConn1 -- _CN_92458761_400000_CN_96107758_400000/RConn3
  T_200511209_400000;275000_Hawthorn_Pit_Substation/LConn1 -- _CN_200511209_400000_CN_43472283_400000/RConn1
  T_200511209_400000;275000_Hawthorn_Pit_Substation/LConn2 -- _CN_200511209_400000_CN_43472283_400000/RConn2
  _CN_200511209_400000_CN_43472283_400000/RConn3 -- T_200511209_400000;275000_Hawthorn_Pit_Substation/LConn3 -- bus185/LConn1
  _CN_142397822_400000_CN_209404646_400000/RConn1 -- T_142397822__/LConn1 -- _CN_142397822_400000_CN_109730296_400000/LConn1
  _CN_142397822_400000_CN_209404646_400000/RConn2 -- T_142397822__/LConn2 -- _CN_142397822_400000_CN_109730296_400000/LConn2
  _CN_142397822_400000_CN_209404646_400000/RConn3 -- T_142397822__/LConn3 -- _CN_142397822_400000_CN_109730296_400000/LConn3 -- bus186/LConn1
  _CN_142397822_400000_CN_109730296_400000/RConn1 -- T_109730296_400000;275000_Lackenby_Substation/LConn1 -- _CN_43472283_400000_CN_109730296_400000/RConn1
  _CN_142397822_400000_CN_109730296_400000/RConn2 -- T_109730296_400000;275000_Lackenby_Substation/LConn2 -- _CN_43472283_400000_CN_109730296_400000/RConn2
  _CN_142397822_400000_CN_109730296_400000/RConn3 -- T_109730296_400000;275000_Lackenby_Substation/LConn3 -- _CN_43472283_400000_CN_109730296_400000/RConn3 -- bus187/LConn1
  West_Thurrock_?_CN_103150854_400000_CN_16582436_400000/RConn1 -- T_16582436_400000;132000_Northfleet_East_Substation/LConn1 -- National_Grid_Northfleet_East_Singlewell_CN_16582436_400000_CN_91010711_400000/LConn1
  West_Thurrock_?_CN_103150854_400000_CN_16582436_400000/RConn2 -- T_16582436_400000;132000_Northfleet_East_Substation/LConn2 -- National_Grid_Northfleet_East_Singlewell_CN_16582436_400000_CN_91010711_400000/LConn2
  West_Thurrock_?_CN_103150854_400000_CN_16582436_400000/RConn3 -- T_16582436_400000;132000_Northfleet_East_Substation/LConn3 -- National_Grid_Northfleet_East_Singlewell_CN_16582436_400000_CN_91010711_400000/LConn3 -- bus188/LConn1
  _CN_34656007_400000_CN_26938722_400000/RConn1 -- T_26938722_400000;132000_Abham_Substation/LConn1 -- _CN_26678829_400000_CN_26938722_400000/RConn1
  _CN_34656007_400000_CN_26938722_400000/RConn2 -- T_26938722_400000;132000_Abham_Substation/LConn2 -- _CN_26678829_400000_CN_26938722_400000/RConn2
  _CN_34656007_400000_CN_26938722_400000/RConn3 -- T_26938722_400000;132000_Abham_Substation/LConn3 -- _CN_26678829_400000_CN_26938722_400000/RConn3 -- bus189/LConn1
  T_88455233__Kingsnorth_Substation/LConn1 -- National_Grid_Kingsnorth_Tilbury_CN_103829261_400000_CN_88455233_400000/RConn1
  T_88455233__Kingsnorth_Substation/LConn2 -- National_Grid_Kingsnorth_Tilbury_CN_103829261_400000_CN_88455233_400000/RConn2
  National_Grid_Kingsnorth_Tilbury_CN_103829261_400000_CN_88455233_400000/RConn3 -- T_88455233__Kingsnorth_Substation/LConn3 -- bus190/LConn1
  T_308653840__/LConn1 -- _CN_308653840_400000_CN_308653841_400000/RConn1
  T_308653840__/LConn2 -- _CN_308653840_400000_CN_308653841_400000/RConn2
  _CN_308653840_400000_CN_308653841_400000/RConn3 -- T_308653840__/LConn3 -- bus191/LConn1
  T_365868376_400000_New_Connahs_Quay_Substation/LConn1 -- _CN_92529432_400000_CN_365868376_400000/RConn1
  T_365868376_400000_New_Connahs_Quay_Substation/LConn2 -- _CN_92529432_400000_CN_365868376_400000/RConn2
  _CN_92529432_400000_CN_365868376_400000/RConn3 -- T_365868376_400000_New_Connahs_Quay_Substation/LConn3 -- bus192/LConn1
  _CN_23059230_400000_CN_30904448_400000/RConn1 -- G_30904448_Didcot_Power_Stations/RConn1 -- National_Grid_Didcot_Bramley_CN_160173033_400000_CN_30904448_400000/LConn1 -- _CN_292470577_400000_CN_30904448_400000/LConn1 -- _CN_263863442_400000_CN_30904448_400000/LConn1
  _CN_23059230_400000_CN_30904448_400000/RConn2 -- G_30904448_Didcot_Power_Stations/RConn2 -- National_Grid_Didcot_Bramley_CN_160173033_400000_CN_30904448_400000/LConn2 -- _CN_292470577_400000_CN_30904448_400000/LConn2 -- _CN_263863442_400000_CN_30904448_400000/LConn2
  _CN_23059230_400000_CN_30904448_400000/RConn3 -- G_30904448_Didcot_Power_Stations/RConn3 -- National_Grid_Didcot_Bramley_CN_160173033_400000_CN_30904448_400000/LConn3 -- bus193/LConn1 -- _CN_292470577_400000_CN_30904448_400000/LConn3 -- _CN_263863442_400000_CN_30904448_400000/LConn3
  _CN_23059230_400000_CN_92340133_400000/RConn1 -- T_92340133_400000;132000_East_Claydon_Substation/LConn1 -- _CN_41710456_400000_CN_92340133_400000/RConn1 -- _CN_90534270_400000_CN_92340133_400000/LConn1
  _CN_23059230_400000_CN_92340133_400000/RConn2 -- T_92340133_400000;132000_East_Claydon_Substation/LConn2 -- _CN_41710456_400000_CN_92340133_400000/RConn2 -- _CN_90534270_400000_CN_92340133_400000/LConn2
  _CN_23059230_400000_CN_92340133_400000/RConn3 -- T_92340133_400000;132000_East_Claydon_Substation/LConn3 -- _CN_41710456_400000_CN_92340133_400000/RConn3 -- _CN_90534270_400000_CN_92340133_400000/LConn3 -- bus194/LConn1
  _CN_38528291_400000_CN_190511290_400000/RConn1 -- T_190511290_400000;132000_/LConn1 -- _CN_190511290_400000_CN_324880597_400000/RConn1
  _CN_38528291_400000_CN_190511290_400000/RConn2 -- T_190511290_400000;132000_/LConn2 -- _CN_190511290_400000_CN_324880597_400000/RConn2
  _CN_38528291_400000_CN_190511290_400000/RConn3 -- T_190511290_400000;132000_/LConn3 -- _CN_190511290_400000_CN_324880597_400000/RConn3 -- bus195/LConn1
  T_91010711_400000;25000_Singlewell_Feeder_Station/LConn1 -- National_Grid_Northfleet_East_Singlewell_CN_16582436_400000_CN_91010711_400000/RConn1
  T_91010711_400000;25000_Singlewell_Feeder_Station/LConn2 -- National_Grid_Northfleet_East_Singlewell_CN_16582436_400000_CN_91010711_400000/RConn2
  National_Grid_Northfleet_East_Singlewell_CN_16582436_400000_CN_91010711_400000/RConn3 -- T_91010711_400000;25000_Singlewell_Feeder_Station/LConn3 -- bus196/LConn1
  T_292470577_400000_Electric_Sub_Station/LConn1 -- _CN_292470577_400000_CN_30904448_400000/RConn1
  T_292470577_400000_Electric_Sub_Station/LConn2 -- _CN_292470577_400000_CN_30904448_400000/RConn2
  _CN_292470577_400000_CN_30904448_400000/RConn3 -- T_292470577_400000_Electric_Sub_Station/LConn3 -- bus197/LConn1
  T_142843255__/LConn1 -- National_Grid_Pentir_Trawsfynydd_CN_98899051_400000_CN_142843255_400000/RConn1
  T_142843255__/LConn2 -- National_Grid_Pentir_Trawsfynydd_CN_98899051_400000_CN_142843255_400000/RConn2
  National_Grid_Pentir_Trawsfynydd_CN_98899051_400000_CN_142843255_400000/RConn3 -- T_142843255__/LConn3 -- bus198/LConn1
  T_280317944__St_Asaph_Substation/LConn1 -- National_Grid_Deeside_Pentir_CN_280317944_400000_CN_290606955_400000/LConn1
  T_280317944__St_Asaph_Substation/LConn2 -- National_Grid_Deeside_Pentir_CN_280317944_400000_CN_290606955_400000/LConn2
  National_Grid_Deeside_Pentir_CN_280317944_400000_CN_290606955_400000/LConn3 -- T_280317944__St_Asaph_Substation/LConn3 -- bus199/LConn1
  T_290606955__/LConn1 -- National_Grid_Deeside_Pentir_CN_280317944_400000_CN_290606955_400000/RConn1
  T_290606955__/LConn2 -- National_Grid_Deeside_Pentir_CN_280317944_400000_CN_290606955_400000/RConn2
  National_Grid_Deeside_Pentir_CN_280317944_400000_CN_290606955_400000/RConn3 -- T_290606955__/LConn3 -- bus200/LConn1
  National_Grid_Melksham_?_CN_103915328_400000_CN_4911067_400000/RConn1 -- G_4911067_Seabank_Power_Station/RConn1 -- _CN_292471784_400000_CN_4911067_400000/LConn1
  National_Grid_Melksham_?_CN_103915328_400000_CN_4911067_400000/RConn2 -- G_4911067_Seabank_Power_Station/RConn2 -- _CN_292471784_400000_CN_4911067_400000/LConn2
  National_Grid_Melksham_?_CN_103915328_400000_CN_4911067_400000/RConn3 -- G_4911067_Seabank_Power_Station/RConn3 -- _CN_292471784_400000_CN_4911067_400000/LConn3 -- bus201/LConn1
  T_193460868__/LConn1 -- _CN_193460868_400000_CN_313495307_400000/RConn1
  T_193460868__/LConn2 -- _CN_193460868_400000_CN_313495307_400000/RConn2
  _CN_193460868_400000_CN_313495307_400000/RConn3 -- T_193460868__/LConn3 -- bus202/LConn1
  T_313180501_400000_/LConn1 -- _CN_313180501_400000_CN_204918278_400000/RConn1
  T_313180501_400000_/LConn2 -- _CN_313180501_400000_CN_204918278_400000/RConn2
  _CN_313180501_400000_CN_204918278_400000/RConn3 -- T_313180501_400000_/LConn3 -- bus203/LConn1
  T_310488541__/LConn1 -- _CN_94004582_400000_CN_310488541_400000/RConn1
  T_310488541__/LConn2 -- _CN_94004582_400000_CN_310488541_400000/RConn2
  _CN_94004582_400000_CN_310488541_400000/RConn3 -- T_310488541__/LConn3 -- bus204/LConn1
  G_310488542_Heysham_Nuclear_Power_Station/RConn1 -- _CN_94004582_400000_CN_310488542_400000/RConn1
  G_310488542_Heysham_Nuclear_Power_Station/RConn2 -- _CN_94004582_400000_CN_310488542_400000/RConn2
  _CN_94004582_400000_CN_310488542_400000/RConn3 -- G_310488542_Heysham_Nuclear_Power_Station/RConn3 -- bus205/LConn1
  T_263863442__Didcot_Substation/LConn1 -- _CN_263863442_400000_CN_30904448_400000/RConn1
  T_263863442__Didcot_Substation/LConn2 -- _CN_263863442_400000_CN_30904448_400000/RConn2
  _CN_263863442_400000_CN_30904448_400000/RConn3 -- T_263863442__Didcot_Substation/LConn3 -- bus206/LConn1
  _CN_92460913_400000_CN_92483460_400000/RConn1 -- T_92483460__/LConn1 -- _CN_92483460_400000_CN_95896505_400000/RConn1
  _CN_92460913_400000_CN_92483460_400000/RConn2 -- T_92483460__/LConn2 -- _CN_92483460_400000_CN_95896505_400000/RConn2
  _CN_92460913_400000_CN_92483460_400000/RConn3 -- T_92483460__/LConn3 -- _CN_92483460_400000_CN_95896505_400000/RConn3 -- bus207/LConn1
  T_88287125_400000;132000_/LConn1 -- _CN_91003253_400000_CN_88287125_400000/RConn1
  T_88287125_400000;132000_/LConn2 -- _CN_91003253_400000_CN_88287125_400000/RConn2
  _CN_91003253_400000_CN_88287125_400000/RConn3 -- T_88287125_400000;132000_/LConn3 -- bus208/LConn1
  _CN_90534270_400000_CN_35287066_400000/RConn1 -- T_90534270_400000;132000_/LConn1 -- _CN_90534270_400000_CN_92340133_400000/RConn1
  _CN_90534270_400000_CN_35287066_400000/RConn2 -- T_90534270_400000;132000_/LConn2 -- _CN_90534270_400000_CN_92340133_400000/RConn2
  _CN_90534270_400000_CN_35287066_400000/RConn3 -- T_90534270_400000;132000_/LConn3 -- _CN_90534270_400000_CN_92340133_400000/RConn3 -- bus209/LConn1
  T_31015820_400000;132000;66000_St_John's_Wood_substation/LConn1 -- The_London_Connection_CN_31015820_400000_CN_371757485_400000/LConn1
  T_31015820_400000;132000;66000_St_John's_Wood_substation/LConn2 -- The_London_Connection_CN_31015820_400000_CN_371757485_400000/LConn2
  The_London_Connection_CN_31015820_400000_CN_371757485_400000/LConn3 -- T_31015820_400000;132000;66000_St_John's_Wood_substation/LConn3 -- bus210/LConn1
  The_London_Connection_CN_31015820_400000_CN_371757485_400000/RConn1 -- T_371757485_400000;275000_/LConn1 -- _CN_371757485_400000_CN_23228362_400000/RConn1
  The_London_Connection_CN_31015820_400000_CN_371757485_400000/RConn2 -- T_371757485_400000;275000_/LConn2 -- _CN_371757485_400000_CN_23228362_400000/RConn2
  The_London_Connection_CN_31015820_400000_CN_371757485_400000/RConn3 -- T_371757485_400000;275000_/LConn3 -- _CN_371757485_400000_CN_23228362_400000/RConn3 -- bus211/LConn1
  T_315965849__/LConn1 -- _CN_315965849_400000_CN_35287066_400000/RConn1
  T_315965849__/LConn2 -- _CN_315965849_400000_CN_35287066_400000/RConn2
  _CN_315965849_400000_CN_35287066_400000/RConn3 -- T_315965849__/LConn3 -- bus212/LConn1
  T_264102298_400000;275000_/LConn1 -- _CN_264102298_400000_CN_88540693_400000/RConn1
  T_264102298_400000;275000_/LConn2 -- _CN_264102298_400000_CN_88540693_400000/RConn2
  _CN_264102298_400000_CN_88540693_400000/RConn3 -- T_264102298_400000;275000_/LConn3 -- bus213/LConn1
  National_Grid_Didcot_Bramley_CN_32796576_400000_CN_160173034_400000/RConn1 -- T_160173034__/LConn1 -- National_Grid_Didcot_Bramley_(underground)_CN_160173033_400000_CN_160173034_400000/LConn1
  National_Grid_Didcot_Bramley_CN_32796576_400000_CN_160173034_400000/RConn2 -- T_160173034__/LConn2 -- National_Grid_Didcot_Bramley_(underground)_CN_160173033_400000_CN_160173034_400000/LConn2
  National_Grid_Didcot_Bramley_CN_32796576_400000_CN_160173034_400000/RConn3 -- T_160173034__/LConn3 -- National_Grid_Didcot_Bramley_(underground)_CN_160173033_400000_CN_160173034_400000/LConn3 -- bus214/LConn1
  T_23167419_400000_/LConn1 -- _CN_23167419_400000_CN_195575988_400000/RConn1
  T_23167419_400000_/LConn2 -- _CN_23167419_400000_CN_195575988_400000/RConn2
  _CN_23167419_400000_CN_195575988_400000/RConn3 -- T_23167419_400000_/LConn3 -- bus215/LConn1
  T_160580052_400000_/LConn1 -- _CN_160580052_400000_CN_34383063_400000/RConn1
  T_160580052_400000_/LConn2 -- _CN_160580052_400000_CN_34383063_400000/RConn2
  _CN_160580052_400000_CN_34383063_400000/RConn3 -- T_160580052_400000_/LConn3 -- bus216/LConn1
  T_292471784_400000;132000_/LConn1 -- _CN_292471784_400000_CN_4911067_400000/RConn1
  T_292471784_400000;132000_/LConn2 -- _CN_292471784_400000_CN_4911067_400000/RConn2
  _CN_292471784_400000_CN_4911067_400000/RConn3 -- T_292471784_400000;132000_/LConn3 -- bus217/LConn1
  National_Grid_Didcot_Bramley_(underground)_CN_160173033_400000_CN_160173034_400000/RConn1 -- T_160173033__/LConn1 -- National_Grid_Didcot_Bramley_CN_160173033_400000_CN_30904448_400000/RConn1
  National_Grid_Didcot_Bramley_(underground)_CN_160173033_400000_CN_160173034_400000/RConn2 -- T_160173033__/LConn2 -- National_Grid_Didcot_Bramley_CN_160173033_400000_CN_30904448_400000/RConn2
  National_Grid_Didcot_Bramley_(underground)_CN_160173033_400000_CN_160173034_400000/RConn3 -- T_160173033__/LConn3 -- National_Grid_Didcot_Bramley_CN_160173033_400000_CN_30904448_400000/RConn3 -- bus218/LConn1
  T_314338799_400000_/LConn1 -- _CN_314338799_400000_CN_324880597_400000/RConn1
  T_314338799_400000_/LConn2 -- _CN_314338799_400000_CN_324880597_400000/RConn2
  _CN_314338799_400000_CN_324880597_400000/RConn3 -- T_314338799_400000_/LConn3 -- bus219/LConn1
  T_143861248_400000_Pembroke_Substation/RConn1 -- L_143861248/LConn1
  T_143861248_400000_Pembroke_Substation/RConn2 -- L_143861248/LConn2
  L_143861248/LConn3 -- T_143861248_400000_Pembroke_Substation/RConn3 -- bus220/LConn1
  T_95749833_400000;275000_CILF_Cilfynydd/RConn1 -- L_95749833/LConn1
  T_95749833_400000;275000_CILF_Cilfynydd/RConn2 -- L_95749833/LConn2
  L_95749833/LConn3 -- T_95749833_400000;275000_CILF_Cilfynydd/RConn3 -- bus221/LConn1
  T_95896505__/RConn1 -- L_95896505/LConn1
  T_95896505__/RConn2 -- L_95896505/LConn2
  L_95896505/LConn3 -- T_95896505__/RConn3 -- bus222/LConn1
  T_95895489_400000_/RConn1 -- L_95895489/LConn1
  T_95895489_400000_/RConn2 -- L_95895489/LConn2
  L_95895489/LConn3 -- T_95895489_400000_/RConn3 -- bus223/LConn1
  T_192220229_400000_Swansea_North_Substation/RConn1 -- L_192220229/LConn1
  T_192220229_400000_Swansea_North_Substation/RConn2 -- L_192220229/LConn2
  L_192220229/LConn3 -- T_192220229_400000_Swansea_North_Substation/RConn3 -- bus224/LConn1
  T_95600440_400000_Swansea_North_Substation/RConn1 -- L_95600440/LConn1
  T_95600440_400000_Swansea_North_Substation/RConn2 -- L_95600440/LConn2
  L_95600440/LConn3 -- T_95600440_400000_Swansea_North_Substation/RConn3 -- bus225/LConn1
  T_51424257__Hinksey_South___Cable_Sealing_End_Compound/RConn1 -- L_51424257/LConn1
  T_51424257__Hinksey_South___Cable_Sealing_End_Compound/RConn2 -- L_51424257/LConn2
  L_51424257/LConn3 -- T_51424257__Hinksey_South___Cable_Sealing_End_Compound/RConn3 -- bus226/LConn1
  T_23059230_400000;132000_Cowley_Substation/RConn1 -- L_23059230/LConn1
  T_23059230_400000;132000_Cowley_Substation/RConn2 -- L_23059230/LConn2
  L_23059230/LConn3 -- T_23059230_400000;132000_Cowley_Substation/RConn3 -- bus227/LConn1
  T_32117744__Hinksey_North___Cable_Sealing_End_Compound/RConn1 -- L_32117744/LConn1
  T_32117744__Hinksey_North___Cable_Sealing_End_Compound/RConn2 -- L_32117744/LConn2
  L_32117744/LConn3 -- T_32117744__Hinksey_North___Cable_Sealing_End_Compound/RConn3 -- bus228/LConn1
  T_376450057_400000_/RConn1 -- L_376450057/LConn1
  T_376450057_400000_/RConn2 -- L_376450057/LConn2
  L_376450057/LConn3 -- T_376450057_400000_/RConn3 -- bus229/LConn1
  T_42799627__Cable_tunnel_shaft/RConn1 -- L_42799627/LConn1
  T_42799627__Cable_tunnel_shaft/RConn2 -- L_42799627/LConn2
  L_42799627/LConn3 -- T_42799627__Cable_tunnel_shaft/RConn3 -- bus230/LConn1
  T_375637875_400000;275000_WHSO_Whitson/RConn1 -- L_375637875/LConn1
  T_375637875_400000;275000_WHSO_Whitson/RConn2 -- L_375637875/LConn2
  L_375637875/LConn3 -- T_375637875_400000;275000_WHSO_Whitson/RConn3 -- bus231/LConn1
  T_42800878_400000_IMPP_Imperial_Park/RConn1 -- L_42800878/LConn1
  T_42800878_400000_IMPP_Imperial_Park/RConn2 -- L_42800878/LConn2
  L_42800878/LConn3 -- T_42800878_400000_IMPP_Imperial_Park/RConn3 -- bus232/LConn1
  T_103962437__Cable_tunnel_shaft/RConn1 -- L_103962437/LConn1
  T_103962437__Cable_tunnel_shaft/RConn2 -- L_103962437/LConn2
  L_103962437/LConn3 -- T_103962437__Cable_tunnel_shaft/RConn3 -- bus233/LConn1
  T_143384076_400000_Strathaven_Substation/RConn1 -- L_143384076/LConn1
  T_143384076_400000_Strathaven_Substation/RConn2 -- L_143384076/LConn2
  L_143384076/LConn3 -- T_143384076_400000_Strathaven_Substation/RConn3 -- bus234/LConn1
  T_143383456_400000;132000_Coalburn_Substation/RConn1 -- L_143383456/LConn1
  T_143383456_400000;132000_Coalburn_Substation/RConn2 -- L_143383456/LConn2
  L_143383456/LConn3 -- T_143383456_400000;132000_Coalburn_Substation/RConn3 -- bus235/LConn1
  T_284874050_400000_/RConn1 -- L_284874050/LConn1
  T_284874050_400000_/RConn2 -- L_284874050/LConn2
  L_284874050/LConn3 -- T_284874050_400000_/RConn3 -- bus236/LConn1
  T_100077745_400000;275000_Kilmarnock_South_Substation/RConn1 -- L_100077745/LConn1
  T_100077745_400000;275000_Kilmarnock_South_Substation/RConn2 -- L_100077745/LConn2
  L_100077745/LConn3 -- T_100077745_400000;275000_Kilmarnock_South_Substation/RConn3 -- bus237/LConn1
  T_308653841__/RConn1 -- L_308653841/LConn1
  T_308653841__/RConn2 -- L_308653841/LConn2
  L_308653841/LConn3 -- T_308653841__/RConn3 -- bus238/LConn1
  T_86071326_400000;275000;132000_Windyhill_Substation/RConn1 -- L_86071326/LConn1
  T_86071326_400000;275000;132000_Windyhill_Substation/RConn2 -- L_86071326/LConn2
  L_86071326/LConn3 -- T_86071326_400000;275000;132000_Windyhill_Substation/RConn3 -- bus239/LConn1
  T_91038272_400000_Inverkip_Substation/RConn1 -- L_91038272/LConn1
  T_91038272_400000_Inverkip_Substation/RConn2 -- L_91038272/LConn2
  L_91038272/LConn3 -- T_91038272_400000_Inverkip_Substation/RConn3 -- bus240/LConn1
  T_143398452_400000_Neilston/RConn1 -- L_143398452/LConn1
  T_143398452_400000_Neilston/RConn2 -- L_143398452/LConn2
  L_143398452/LConn3 -- T_143398452_400000_Neilston/RConn3 -- bus241/LConn1
  T_308653843_400000_/RConn1 -- L_308653843/LConn1
  T_308653843_400000_/RConn2 -- L_308653843/LConn2
  L_308653843/LConn3 -- T_308653843_400000_/RConn3 -- bus242/LConn1
  T_96905262_400000;275000_/RConn1 -- L_96905262/LConn1
  T_96905262_400000;275000_/RConn2 -- L_96905262/LConn2
  L_96905262/LConn3 -- T_96905262_400000;275000_/RConn3 -- bus243/LConn1
  T_262532045_400000_/RConn1 -- L_262532045/LConn1
  T_262532045_400000_/RConn2 -- L_262532045/LConn2
  L_262532045/LConn3 -- T_262532045_400000_/RConn3 -- bus244/LConn1
  T_262523325_400000;132000_/RConn1 -- L_262523325/LConn1
  T_262523325_400000;132000_/RConn2 -- L_262523325/LConn2
  L_262523325/LConn3 -- T_262523325_400000;132000_/RConn3 -- bus245/LConn1
  T_97551518__/RConn1 -- L_97551518/LConn1
  T_97551518__/RConn2 -- L_97551518/LConn2
  L_97551518/LConn3 -- T_97551518__/RConn3 -- bus246/LConn1
  T_77065229_400000;132000_Stocking_Pelham_Substation/RConn1 -- L_77065229/LConn1
  T_77065229_400000;132000_Stocking_Pelham_Substation/RConn2 -- L_77065229/LConn2
  L_77065229/LConn3 -- T_77065229_400000;132000_Stocking_Pelham_Substation/RConn3 -- bus247/LConn1
  T_264650844_400000_/RConn1 -- L_264650844/LConn1
  T_264650844_400000_/RConn2 -- L_264650844/LConn2
  L_264650844/LConn3 -- T_264650844_400000_/RConn3 -- bus248/LConn1
  T_25422135_400000;132000_Bramford_Substation/RConn1 -- L_25422135/LConn1
  T_25422135_400000;132000_Bramford_Substation/RConn2 -- L_25422135/LConn2
  L_25422135/LConn3 -- T_25422135_400000;132000_Bramford_Substation/RConn3 -- bus249/LConn1
  T_29111908_400000;132000_Braintree_Substation/RConn1 -- L_29111908/LConn1
  T_29111908_400000;132000_Braintree_Substation/RConn2 -- L_29111908/LConn2
  L_29111908/LConn3 -- T_29111908_400000;132000_Braintree_Substation/RConn3 -- bus250/LConn1
  T_29111844_400000;132000_Rayleigh_Main_Substation/RConn1 -- L_29111844/LConn1
  T_29111844_400000;132000_Rayleigh_Main_Substation/RConn2 -- L_29111844/LConn2
  L_29111844/LConn3 -- T_29111844_400000;132000_Rayleigh_Main_Substation/RConn3 -- bus251/LConn1
  T_25935453_400000;132000_Burwell_Main_Substation_(BURW)/RConn1 -- L_25935453/LConn1
  T_25935453_400000;132000_Burwell_Main_Substation_(BURW)/RConn2 -- L_25935453/LConn2
  L_25935453/LConn3 -- T_25935453_400000;132000_Burwell_Main_Substation_(BURW)/RConn3 -- bus252/LConn1
  T_38528291_400000;132000_Walpole_Substation/RConn1 -- L_38528291/LConn1
  T_38528291_400000;132000_Walpole_Substation/RConn2 -- L_38528291/LConn2
  L_38528291/LConn3 -- T_38528291_400000;132000_Walpole_Substation/RConn3 -- bus253/LConn1
  T_25385285__Rye_House_Substation/RConn1 -- L_25385285/LConn1
  T_25385285__Rye_House_Substation/RConn2 -- L_25385285/LConn2
  L_25385285/LConn3 -- T_25385285__Rye_House_Substation/RConn3 -- bus254/LConn1
  T_22975329_400000;275000_Waltham_Cross_Substation/RConn1 -- L_22975329/LConn1
  T_22975329_400000;275000_Waltham_Cross_Substation/RConn2 -- L_22975329/LConn2
  L_22975329/LConn3 -- T_22975329_400000;275000_Waltham_Cross_Substation/RConn3 -- bus255/LConn1
  T_24165071_400000_Wymondley_Substation/RConn1 -- L_24165071/LConn1
  T_24165071_400000_Wymondley_Substation/RConn2 -- L_24165071/LConn2
  L_24165071/LConn3 -- T_24165071_400000_Wymondley_Substation/RConn3 -- bus256/LConn1
  T_97256377_400000;275000_/RConn1 -- L_97256377/LConn1
  T_97256377_400000;275000_/RConn2 -- L_97256377/LConn2
  L_97256377/LConn3 -- T_97256377_400000;275000_/RConn3 -- bus257/LConn1
  T_81048391_400000;275000;132000_Penwortham_Substation/RConn1 -- L_81048391/LConn1
  T_81048391_400000;275000;132000_Penwortham_Substation/RConn2 -- L_81048391/LConn2
  L_81048391/LConn3 -- T_81048391_400000;275000;132000_Penwortham_Substation/RConn3 -- bus258/LConn1
  T_55578199_400000_Padiham_Substation/RConn1 -- L_55578199/LConn1
  T_55578199_400000_Padiham_Substation/RConn2 -- L_55578199/LConn2
  L_55578199/LConn3 -- T_55578199_400000_Padiham_Substation/RConn3 -- bus259/LConn1
  T_92529432_400000_Daines_Substation/RConn1 -- L_92529432/LConn1
  T_92529432_400000_Daines_Substation/RConn2 -- L_92529432/LConn2
  L_92529432/LConn3 -- T_92529432_400000_Daines_Substation/RConn3 -- bus260/LConn1
  T_92676046_400000;132000_/RConn1 -- L_92676046/LConn1
  T_92676046_400000;132000_/RConn2 -- L_92676046/LConn2
  L_92676046/LConn3 -- T_92676046_400000;132000_/RConn3 -- bus261/LConn1
  T_92737152_400000_/RConn1 -- L_92737152/LConn1
  T_92737152_400000_/RConn2 -- L_92737152/LConn2
  L_92737152/LConn3 -- T_92737152_400000_/RConn3 -- bus262/LConn1
  T_293584682__/RConn1 -- L_293584682/LConn1
  T_293584682__/RConn2 -- L_293584682/LConn2
  L_293584682/LConn3 -- T_293584682__/RConn3 -- bus263/LConn1
  T_159038999_400000_/RConn1 -- L_159038999/LConn1
  T_159038999_400000_/RConn2 -- L_159038999/LConn2
  L_159038999/LConn3 -- T_159038999_400000_/RConn3 -- bus264/LConn1
  T_291629706__/RConn1 -- L_291629706/LConn1
  T_291629706__/RConn2 -- L_291629706/LConn2
  L_291629706/LConn3 -- T_291629706__/RConn3 -- bus265/LConn1
  T_90539508_400000_/RConn1 -- L_90539508/LConn1
  T_90539508_400000_/RConn2 -- L_90539508/LConn2
  L_90539508/LConn3 -- T_90539508_400000_/RConn3 -- bus266/LConn1
  T_101077623_400000;275000_/RConn1 -- L_101077623/LConn1
  T_101077623_400000;275000_/RConn2 -- L_101077623/LConn2
  L_101077623/LConn3 -- T_101077623_400000;275000_/RConn3 -- bus267/LConn1
  T_313495303__/RConn1 -- L_313495303/LConn1
  T_313495303__/RConn2 -- L_313495303/LConn2
  L_313495303/LConn3 -- T_313495303__/RConn3 -- bus268/LConn1
  T_90547679_400000_/RConn1 -- L_90547679/LConn1
  T_90547679_400000_/RConn2 -- L_90547679/LConn2
  L_90547679/LConn3 -- T_90547679_400000_/RConn3 -- bus269/LConn1
  T_102198808_400000;132000_Eccles_Substation/RConn1 -- L_102198808/LConn1
  T_102198808_400000;132000_Eccles_Substation/RConn2 -- L_102198808/LConn2
  L_102198808/LConn3 -- T_102198808_400000;132000_Eccles_Substation/RConn3 -- bus270/LConn1
  T_308788887_400000_/RConn1 -- L_308788887/LConn1
  T_308788887_400000_/RConn2 -- L_308788887/LConn2
  L_308788887/LConn3 -- T_308788887_400000_/RConn3 -- bus271/LConn1
  T_310502642_400000;275000_/RConn1 -- L_310502642/LConn1
  T_310502642_400000;275000_/RConn2 -- L_310502642/LConn2
  L_310502642/LConn3 -- T_310502642_400000;275000_/RConn3 -- bus272/LConn1
  T_91955171_400000;275000;132000_Stella_West_Sub_Station/RConn1 -- L_91955171/LConn1
  T_91955171_400000;275000;132000_Stella_West_Sub_Station/RConn2 -- L_91955171/LConn2
  L_91955171/LConn3 -- T_91955171_400000;275000;132000_Stella_West_Sub_Station/RConn3 -- bus273/LConn1
  T_97551523__/RConn1 -- L_97551523/LConn1
  T_97551523__/RConn2 -- L_97551523/LConn2
  L_97551523/LConn3 -- T_97551523__/RConn3 -- bus274/LConn1
  T_314338845__/RConn1 -- L_314338845/LConn1
  T_314338845__/RConn2 -- L_314338845/LConn2
  L_314338845/LConn3 -- T_314338845__/RConn3 -- bus275/LConn1
  T_143905069_400000;275000_High_Marnham_Substation/RConn1 -- L_143905069/LConn1
  T_143905069_400000;275000_High_Marnham_Substation/RConn2 -- L_143905069/LConn2
  L_143905069/LConn3 -- T_143905069_400000;275000_High_Marnham_Substation/RConn3 -- bus276/LConn1
  T_91003253_400000;132000_Staythorpe_Substation/RConn1 -- L_91003253/LConn1
  T_91003253_400000;132000_Staythorpe_Substation/RConn2 -- L_91003253/LConn2
  L_91003253/LConn3 -- T_91003253_400000;132000_Staythorpe_Substation/RConn3 -- bus277/LConn1
  T_314338790_400000_/RConn1 -- L_314338790/LConn1
  T_314338790_400000_/RConn2 -- L_314338790/LConn2
  L_314338790/LConn3 -- T_314338790_400000_/RConn3 -- bus278/LConn1
  T_314338851__/RConn1 -- L_314338851/LConn1
  T_314338851__/RConn2 -- L_314338851/LConn2
  L_314338851/LConn3 -- T_314338851__/RConn3 -- bus279/LConn1
  T_314338849__/RConn1 -- L_314338849/LConn1
  T_314338849__/RConn2 -- L_314338849/LConn2
  L_314338849/LConn3 -- T_314338849__/RConn3 -- bus280/LConn1
  T_310495264_400000;132000_Stanah_Substation/RConn1 -- L_310495264/LConn1
  T_310495264_400000;132000_Stanah_Substation/RConn2 -- L_310495264/LConn2
  L_310495264/LConn3 -- T_310495264_400000;132000_Stanah_Substation/RConn3 -- bus281/LConn1
  T_94004582_400000_Heysham_Substation/RConn1 -- L_94004582/LConn1
  T_94004582_400000_Heysham_Substation/RConn2 -- L_94004582/LConn2
  L_94004582/LConn3 -- T_94004582_400000_Heysham_Substation/RConn3 -- bus282/LConn1
  T_100773252_400000_/RConn1 -- L_100773252/LConn1
  T_100773252_400000_/RConn2 -- L_100773252/LConn2
  L_100773252/LConn3 -- T_100773252_400000_/RConn3 -- bus283/LConn1
  T_94530230_400000;275000_Tilbury_Substation/RConn1 -- L_94530230/LConn1
  T_94530230_400000;275000_Tilbury_Substation/RConn2 -- L_94530230/LConn2
  L_94530230/LConn3 -- T_94530230_400000;275000_Tilbury_Substation/RConn3 -- bus284/LConn1
  T_264214748__/RConn1 -- L_264214748/LConn1
  T_264214748__/RConn2 -- L_264214748/LConn2
  L_264214748/LConn3 -- T_264214748__/RConn3 -- bus285/LConn1
  T_164380199_400000;132000_Elland_Substation/RConn1 -- L_164380199/LConn1
  T_164380199_400000;132000_Elland_Substation/RConn2 -- L_164380199/LConn2
  L_164380199/LConn3 -- T_164380199_400000;132000_Elland_Substation/RConn3 -- bus286/LConn1
  T_193460871__/RConn1 -- L_193460871/LConn1
  T_193460871__/RConn2 -- L_193460871/LConn2
  L_193460871/LConn3 -- T_193460871__/RConn3 -- bus287/LConn1
  T_193617444_400000_Ferrybridge_C_275kV_Substation/RConn1 -- L_193617444/LConn1
  T_193617444_400000_Ferrybridge_C_275kV_Substation/RConn2 -- L_193617444/LConn2
  L_193617444/LConn3 -- T_193617444_400000_Ferrybridge_C_275kV_Substation/RConn3 -- bus288/LConn1
  T_163036722_400000_/RConn1 -- L_163036722/LConn1
  T_163036722_400000_/RConn2 -- L_163036722/LConn2
  L_163036722/LConn3 -- T_163036722_400000_/RConn3 -- bus289/LConn1
  T_292220969_400000_/RConn1 -- L_292220969/LConn1
  T_292220969_400000_/RConn2 -- L_292220969/LConn2
  L_292220969/LConn3 -- T_292220969_400000_/RConn3 -- bus290/LConn1
  T_143791249_400000;132000_Indian_Queens_Substation/RConn1 -- L_143791249/LConn1
  T_143791249_400000;132000_Indian_Queens_Substation/RConn2 -- L_143791249/LConn2
  L_143791249/LConn3 -- T_143791249_400000;132000_Indian_Queens_Substation/RConn3 -- bus291/LConn1
  T_109189895__/RConn1 -- L_109189895/LConn1
  T_109189895__/RConn2 -- L_109189895/LConn2
  L_109189895/LConn3 -- T_109189895__/RConn3 -- bus292/LConn1
  T_109189893__/RConn1 -- L_109189893/LConn1
  T_109189893__/RConn2 -- L_109189893/LConn2
  L_109189893/LConn3 -- T_109189893__/RConn3 -- bus293/LConn1
  T_23988786_400000_Nursling_Substation/RConn1 -- L_23988786/LConn1
  T_23988786_400000_Nursling_Substation/RConn2 -- L_23988786/LConn2
  L_23988786/LConn3 -- T_23988786_400000_Nursling_Substation/RConn3 -- bus294/LConn1
  T_20851038_400000;132000_Lovedean_Substation/RConn1 -- L_20851038/LConn1
  T_20851038_400000;132000_Lovedean_Substation/RConn2 -- L_20851038/LConn2
  L_20851038/LConn3 -- T_20851038_400000;132000_Lovedean_Substation/RConn3 -- bus295/LConn1
  T_5728891_400000_Fawley_Substation/RConn1 -- L_5728891/LConn1
  T_5728891_400000_Fawley_Substation/RConn2 -- L_5728891/LConn2
  L_5728891/LConn3 -- T_5728891_400000_Fawley_Substation/RConn3 -- bus296/LConn1
  T_90099036_400000;132000_Mannington_Substation/RConn1 -- L_90099036/LConn1
  T_90099036_400000;132000_Mannington_Substation/RConn2 -- L_90099036/LConn2
  L_90099036/LConn3 -- T_90099036_400000;132000_Mannington_Substation/RConn3 -- bus297/LConn1
  T_292372019_400000_/RConn1 -- L_292372019/LConn1
  T_292372019_400000_/RConn2 -- L_292372019/LConn2
  L_292372019/LConn3 -- T_292372019_400000_/RConn3 -- bus298/LConn1
  T_103915328_400000;275000;132000_Melksham_Substation/RConn1 -- L_103915328/LConn1
  T_103915328_400000;275000;132000_Melksham_Substation/RConn2 -- L_103915328/LConn2
  L_103915328/LConn3 -- T_103915328_400000;275000;132000_Melksham_Substation/RConn3 -- bus299/LConn1
  T_119616836_400000;132000_Taunton_Substation/RConn1 -- L_119616836/LConn1
  T_119616836_400000;132000_Taunton_Substation/RConn2 -- L_119616836/LConn2
  L_119616836/LConn3 -- T_119616836_400000;132000_Taunton_Substation/RConn3 -- bus300/LConn1
  T_304620087_400000_/RConn1 -- L_304620087/LConn1
  T_304620087_400000_/RConn2 -- L_304620087/LConn2
  L_304620087/LConn3 -- T_304620087_400000_/RConn3 -- bus301/LConn1
  T_102549055_400000;275000_/RConn1 -- L_102549055/LConn1
  T_102549055_400000;275000_/RConn2 -- L_102549055/LConn2
  L_102549055/LConn3 -- T_102549055_400000;275000_/RConn3 -- bus302/LConn1
  T_103150854_400000;275000_West_Thurrock_Substation/RConn1 -- L_103150854/LConn1
  T_103150854_400000;275000_West_Thurrock_Substation/RConn2 -- L_103150854/LConn2
  L_103150854/LConn3 -- T_103150854_400000;275000_West_Thurrock_Substation/RConn3 -- bus303/LConn1
  T_23228362_400000_West_Ham_Substation/RConn1 -- L_23228362/LConn1
  T_23228362_400000_West_Ham_Substation/RConn2 -- L_23228362/LConn2
  L_23228362/LConn3 -- T_23228362_400000_West_Ham_Substation/RConn3 -- bus304/LConn1
  T_23281217_400000_Sellindge_Converter_Station/RConn1 -- L_23281217/LConn1
  T_23281217_400000_Sellindge_Converter_Station/RConn2 -- L_23281217/LConn2
  L_23281217/LConn3 -- T_23281217_400000_Sellindge_Converter_Station/RConn3 -- bus305/LConn1
  T_87953830_400000_Canterbury_North_Substation/RConn1 -- L_87953830/LConn1
  T_87953830_400000_Canterbury_North_Substation/RConn2 -- L_87953830/LConn2
  L_87953830/LConn3 -- T_87953830_400000_Canterbury_North_Substation/RConn3 -- bus306/LConn1
  T_49922626_400000;132000_Chickerell_Substation/RConn1 -- L_49922626/LConn1
  T_49922626_400000;132000_Chickerell_Substation/RConn2 -- L_49922626/LConn2
  L_49922626/LConn3 -- T_49922626_400000;132000_Chickerell_Substation/RConn3 -- bus307/LConn1
  T_26678829_400000;132000_Exeter_Substation/RConn1 -- L_26678829/LConn1
  T_26678829_400000;132000_Exeter_Substation/RConn2 -- L_26678829/LConn2
  L_26678829/LConn3 -- T_26678829_400000;132000_Exeter_Substation/RConn3 -- bus308/LConn1
  T_34205588_400000;132000_Axminster_Substation/RConn1 -- L_34205588/LConn1
  T_34205588_400000;132000_Axminster_Substation/RConn2 -- L_34205588/LConn2
  L_34205588/LConn3 -- T_34205588_400000;132000_Axminster_Substation/RConn3 -- bus309/LConn1
  T_264104518_400000;132000_Cleve_Hill_Substation/RConn1 -- L_264104518/LConn1
  T_264104518_400000;132000_Cleve_Hill_Substation/RConn2 -- L_264104518/LConn2
  L_264104518/LConn3 -- T_264104518_400000;132000_Cleve_Hill_Substation/RConn3 -- bus310/LConn1
  T_91010022_400000;132000_Kemsley_Substation/RConn1 -- L_91010022/LConn1
  T_91010022_400000;132000_Kemsley_Substation/RConn2 -- L_91010022/LConn2
  L_91010022/LConn3 -- T_91010022_400000;132000_Kemsley_Substation/RConn3 -- bus311/LConn1
  T_23299657_400000_Rowdown_Substation/RConn1 -- L_23299657/LConn1
  T_23299657_400000_Rowdown_Substation/RConn2 -- L_23299657/LConn2
  L_23299657/LConn3 -- T_23299657_400000_Rowdown_Substation/RConn3 -- bus312/LConn1
  T_93878866__/RConn1 -- L_93878866/LConn1
  T_93878866__/RConn2 -- L_93878866/LConn2
  L_93878866/LConn3 -- T_93878866__/RConn3 -- bus313/LConn1
  T_293585871__/RConn1 -- L_293585871/LConn1
  T_293585871__/RConn2 -- L_293585871/LConn2
  L_293585871/LConn3 -- T_293585871__/RConn3 -- bus314/LConn1
  T_93878867_400000;132000_/RConn1 -- L_93878867/LConn1
  T_93878867_400000;132000_/RConn2 -- L_93878867/LConn2
  L_93878867/LConn3 -- T_93878867_400000;132000_/RConn3 -- bus315/LConn1
  T_41809491_400000_Sundon_Substation/RConn1 -- L_41809491/LConn1
  T_41809491_400000_Sundon_Substation/RConn2 -- L_41809491/LConn2
  L_41809491/LConn3 -- T_41809491_400000_Sundon_Substation/RConn3 -- bus316/LConn1
  T_89453364_400000_/RConn1 -- L_89453364/LConn1
  T_89453364_400000_/RConn2 -- L_89453364/LConn2
  L_89453364/LConn3 -- T_89453364_400000_/RConn3 -- bus317/LConn1
  T_4746208_400000;275000;132000_Elstree_Substation/RConn1 -- L_4746208/LConn1
  T_4746208_400000;275000;132000_Elstree_Substation/RConn2 -- L_4746208/LConn2
  L_4746208/LConn3 -- T_4746208_400000;275000;132000_Elstree_Substation/RConn3 -- bus318/LConn1
  T_142841192_400000;275000;132000_Bradford_West_Substation/RConn1 -- L_142841192/LConn1
  T_142841192_400000;275000;132000_Bradford_West_Substation/RConn2 -- L_142841192/LConn2
  L_142841192/LConn3 -- T_142841192_400000;275000;132000_Bradford_West_Substation/RConn3 -- bus319/LConn1
  T_90547674_400000;275000_Monk_Fryston_substation/RConn1 -- L_90547674/LConn1
  T_90547674_400000;275000_Monk_Fryston_substation/RConn2 -- L_90547674/LConn2
  L_90547674/LConn3 -- T_90547674_400000;275000_Monk_Fryston_substation/RConn3 -- bus320/LConn1
  T_143219044_400000;132000_Gretna_Substation/RConn1 -- L_143219044/LConn1
  T_143219044_400000;132000_Gretna_Substation/RConn2 -- L_143219044/LConn2
  L_143219044/LConn3 -- T_143219044_400000;132000_Gretna_Substation/RConn3 -- bus321/LConn1
  T_88799419_400000;275000;132000_Harker_Substation/RConn1 -- L_88799419/LConn1
  T_88799419_400000;275000;132000_Harker_Substation/RConn2 -- L_88799419/LConn2
  L_88799419/LConn3 -- T_88799419_400000;275000;132000_Harker_Substation/RConn3 -- bus322/LConn1
  T_100861711_400000_Keadby_400kV_Substation/RConn1 -- L_100861711/LConn1
  T_100861711_400000_Keadby_400kV_Substation/RConn2 -- L_100861711/LConn2
  L_100861711/LConn3 -- T_100861711_400000_Keadby_400kV_Substation/RConn3 -- bus323/LConn1
  T_159736514_400000;275000_Brinsworth_Switching_Station/RConn1 -- L_159736514/LConn1
  T_159736514_400000;275000_Brinsworth_Switching_Station/RConn2 -- L_159736514/LConn2
  L_159736514/LConn3 -- T_159736514_400000;275000_Brinsworth_Switching_Station/RConn3 -- bus324/LConn1
  T_257311344_400000;132000_/RConn1 -- L_257311344/LConn1
  T_257311344_400000;132000_/RConn2 -- L_257311344/LConn2
  L_257311344/LConn3 -- T_257311344_400000;132000_/RConn3 -- bus325/LConn1
  T_160279525_400000;132000_Grimsby_West_Substation/RConn1 -- L_160279525/LConn1
  T_160279525_400000;132000_Grimsby_West_Substation/RConn2 -- L_160279525/LConn2
  L_160279525/LConn3 -- T_160279525_400000;132000_Grimsby_West_Substation/RConn3 -- bus326/LConn1
  T_205132633_400000_/RConn1 -- L_205132633/LConn1
  T_205132633_400000_/RConn2 -- L_205132633/LConn2
  L_205132633/LConn3 -- T_205132633_400000_/RConn3 -- bus327/LConn1
  T_33917128_400000;275000;132000_Creyke_Beck_Substation/RConn1 -- L_33917128/LConn1
  T_33917128_400000;275000;132000_Creyke_Beck_Substation/RConn2 -- L_33917128/LConn2
  L_33917128/LConn3 -- T_33917128_400000;275000;132000_Creyke_Beck_Substation/RConn3 -- bus328/LConn1
  T_264650878__/RConn1 -- L_264650878/LConn1
  T_264650878__/RConn2 -- L_264650878/LConn2
  L_264650878/LConn3 -- T_264650878__/RConn3 -- bus329/LConn1
  T_143783006_400000_/RConn1 -- L_143783006/LConn1
  T_143783006_400000_/RConn2 -- L_143783006/LConn2
  L_143783006/LConn3 -- T_143783006_400000_/RConn3 -- bus330/LConn1
  T_28691559_400000;132000_Ninfield_Substation/RConn1 -- L_28691559/LConn1
  T_28691559_400000;132000_Ninfield_Substation/RConn2 -- L_28691559/LConn2
  L_28691559/LConn3 -- T_28691559_400000;132000_Ninfield_Substation/RConn3 -- bus331/LConn1
  T_91082448_400000;132000_Bolney_Substation/RConn1 -- L_91082448/LConn1
  T_91082448_400000;132000_Bolney_Substation/RConn2 -- L_91082448/LConn2
  L_91082448/LConn3 -- T_91082448_400000;132000_Bolney_Substation/RConn3 -- bus332/LConn1
  T_25629803_400000_Thornton_Substation/RConn1 -- L_25629803/LConn1
  T_25629803_400000_Thornton_Substation/RConn2 -- L_25629803/LConn2
  L_25629803/LConn3 -- T_25629803_400000_Thornton_Substation/RConn3 -- bus333/LConn1
  T_90125443_400000_/RConn1 -- L_90125443/LConn1
  T_90125443_400000_/RConn2 -- L_90125443/LConn2
  L_90125443/LConn3 -- T_90125443_400000_/RConn3 -- bus334/LConn1
  T_209404646__/RConn1 -- L_209404646/LConn1
  T_209404646__/RConn2 -- L_209404646/LConn2
  L_209404646/LConn3 -- T_209404646__/RConn3 -- bus335/LConn1
  T_45357172_400000;132000_Hutton_Substation/RConn1 -- L_45357172/LConn1
  T_45357172_400000;132000_Hutton_Substation/RConn2 -- L_45357172/LConn2
  L_45357172/LConn3 -- T_45357172_400000;132000_Hutton_Substation/RConn3 -- bus336/LConn1
  T_88389243_400000;132000_Fleet_Substation/RConn1 -- L_88389243/LConn1
  T_88389243_400000;132000_Fleet_Substation/RConn2 -- L_88389243/LConn2
  L_88389243/LConn3 -- T_88389243_400000;132000_Fleet_Substation/RConn3 -- bus337/LConn1
  T_32796576_400000;132000_Bramley_Substation/RConn1 -- L_32796576/LConn1
  T_32796576_400000;132000_Bramley_Substation/RConn2 -- L_32796576/LConn2
  L_32796576/LConn3 -- T_32796576_400000;132000_Bramley_Substation/RConn3 -- bus338/LConn1
  T_293585872__/RConn1 -- L_293585872/LConn1
  T_293585872__/RConn2 -- L_293585872/LConn2
  L_293585872/LConn3 -- T_293585872__/RConn3 -- bus339/LConn1
  T_264650881__/RConn1 -- L_264650881/LConn1
  T_264650881__/RConn2 -- L_264650881/LConn2
  L_264650881/LConn3 -- T_264650881__/RConn3 -- bus340/LConn1
  T_32227788_400000_Norwich_Main_Substation/RConn1 -- L_32227788/LConn1
  T_32227788_400000_Norwich_Main_Substation/RConn2 -- L_32227788/LConn2
  L_32227788/LConn3 -- T_32227788_400000_Norwich_Main_Substation/RConn3 -- bus341/LConn1
  T_144135298_400000;275000_West_Weybridge_Substation/RConn1 -- L_144135298/LConn1
  T_144135298_400000;275000_West_Weybridge_Substation/RConn2 -- L_144135298/LConn2
  L_144135298/LConn3 -- T_144135298_400000;275000_West_Weybridge_Substation/RConn3 -- bus342/LConn1
  T_43472283_400000;132000_Norton_Sub_Station/RConn1 -- L_43472283/LConn1
  T_43472283_400000;132000_Norton_Sub_Station/RConn2 -- L_43472283/LConn2
  L_43472283/LConn3 -- T_43472283_400000;132000_Norton_Sub_Station/RConn3 -- bus343/LConn1
  T_94583940__/RConn1 -- L_94583940/LConn1
  T_94583940__/RConn2 -- L_94583940/LConn2
  L_94583940/LConn3 -- T_94583940__/RConn3 -- bus344/LConn1
  T_23167368_400000_Connahs_Quay_Substation/RConn1 -- L_23167368/LConn1
  T_23167368_400000_Connahs_Quay_Substation/RConn2 -- L_23167368/LConn2
  L_23167368/LConn3 -- T_23167368_400000_Connahs_Quay_Substation/RConn3 -- bus345/LConn1
  T_23309078_400000_Chilling_Substation/RConn1 -- L_23309078/LConn1
  T_23309078_400000_Chilling_Substation/RConn2 -- L_23309078/LConn2
  L_23309078/LConn3 -- T_23309078_400000_Chilling_Substation/RConn3 -- bus346/LConn1
  T_23300984_400000_Chilling_Substation/RConn1 -- L_23300984/LConn1
  T_23300984_400000_Chilling_Substation/RConn2 -- L_23300984/LConn2
  L_23300984/LConn3 -- T_23300984_400000_Chilling_Substation/RConn3 -- bus347/LConn1
  T_142738881__/RConn1 -- L_142738881/LConn1
  T_142738881__/RConn2 -- L_142738881/LConn2
  L_142738881/LConn3 -- T_142738881__/RConn3 -- bus348/LConn1
  T_142738882__/RConn1 -- L_142738882/LConn1
  T_142738882__/RConn2 -- L_142738882/LConn2
  L_142738882/LConn3 -- T_142738882__/RConn3 -- bus349/LConn1
  T_147672722_400000_/RConn1 -- L_147672722/LConn1
  T_147672722_400000_/RConn2 -- L_147672722/LConn2
  L_147672722/LConn3 -- T_147672722_400000_/RConn3 -- bus350/LConn1
  T_100009331_400000;132000_Alverdiscott_Substation/RConn1 -- L_100009331/LConn1
  T_100009331_400000;132000_Alverdiscott_Substation/RConn2 -- L_100009331/LConn2
  L_100009331/LConn3 -- T_100009331_400000;132000_Alverdiscott_Substation/RConn3 -- bus351/LConn1
  T_34656007_400000;132000_Landulph_Substation/RConn1 -- L_34656007/LConn1
  T_34656007_400000;132000_Landulph_Substation/RConn2 -- L_34656007/LConn2
  L_34656007/LConn3 -- T_34656007_400000;132000_Landulph_Substation/RConn3 -- bus352/LConn1
  T_95159241_400000;275000_/RConn1 -- L_95159241/LConn1
  T_95159241_400000;275000_/RConn2 -- L_95159241/LConn2
  L_95159241/LConn3 -- T_95159241_400000;275000_/RConn3 -- bus353/LConn1
  T_89427607_400000_Transformer_House/RConn1 -- L_89427607/LConn1
  T_89427607_400000_Transformer_House/RConn2 -- L_89427607/LConn2
  L_89427607/LConn3 -- T_89427607_400000_Transformer_House/RConn3 -- bus354/LConn1
  T_98899051_400000;132000_Pentir_Substation/RConn1 -- L_98899051/LConn1
  T_98899051_400000;132000_Pentir_Substation/RConn2 -- L_98899051/LConn2
  L_98899051/LConn3 -- T_98899051_400000;132000_Pentir_Substation/RConn3 -- bus355/LConn1
  T_220798107_400000;132000_Spennymoor_Substation/RConn1 -- L_220798107/LConn1
  T_220798107_400000;132000_Spennymoor_Substation/RConn2 -- L_220798107/LConn2
  L_220798107/LConn3 -- T_220798107_400000;132000_Spennymoor_Substation/RConn3 -- bus356/LConn1
  T_87204522_400000;275000;132000_Drakelow_Substation/RConn1 -- L_87204522/LConn1
  T_87204522_400000;275000;132000_Drakelow_Substation/RConn2 -- L_87204522/LConn2
  L_87204522/LConn3 -- T_87204522_400000;275000;132000_Drakelow_Substation/RConn3 -- bus357/LConn1
  T_221490974__/RConn1 -- L_221490974/LConn1
  T_221490974__/RConn2 -- L_221490974/LConn2
  L_221490974/LConn3 -- T_221490974__/RConn3 -- bus358/LConn1
  T_277887478_400000_Willington_Substation/RConn1 -- L_277887478/LConn1
  T_277887478_400000_Willington_Substation/RConn2 -- L_277887478/LConn2
  L_277887478/LConn3 -- T_277887478_400000_Willington_Substation/RConn3 -- bus359/LConn1
  T_49499923_400000;275000_Hams_Hall_Substation/RConn1 -- L_49499923/LConn1
  T_49499923_400000;275000_Hams_Hall_Substation/RConn2 -- L_49499923/LConn2
  L_49499923/LConn3 -- T_49499923_400000;275000_Hams_Hall_Substation/RConn3 -- bus360/LConn1
  T_167621580_400000;275000;132000_/RConn1 -- L_167621580/LConn1
  T_167621580_400000;275000;132000_/RConn2 -- L_167621580/LConn2
  L_167621580/LConn3 -- T_167621580_400000;275000;132000_/RConn3 -- bus361/LConn1
  T_87207123_400000;132000_Cellarhead_Substation/RConn1 -- L_87207123/LConn1
  T_87207123_400000;132000_Cellarhead_Substation/RConn2 -- L_87207123/LConn2
  L_87207123/LConn3 -- T_87207123_400000;132000_Cellarhead_Substation/RConn3 -- bus362/LConn1
  T_142741752_400000_/RConn1 -- L_142741752/LConn1
  T_142741752_400000_/RConn2 -- L_142741752/LConn2
  L_142741752/LConn3 -- T_142741752_400000_/RConn3 -- bus363/LConn1
  T_165506012_400000_/RConn1 -- L_165506012/LConn1
  T_165506012_400000_/RConn2 -- L_165506012/LConn2
  L_165506012/LConn3 -- T_165506012_400000_/RConn3 -- bus364/LConn1
  T_92458761_400000;132000_Penn_Substation/RConn1 -- L_92458761/LConn1
  T_92458761_400000;132000_Penn_Substation/RConn2 -- L_92458761/LConn2
  L_92458761/LConn3 -- T_92458761_400000;132000_Penn_Substation/RConn3 -- bus365/LConn1
  T_92419253_400000_Macclesfield_Substation/RConn1 -- L_92419253/LConn1
  T_92419253_400000_Macclesfield_Substation/RConn2 -- L_92419253/LConn2
  L_92419253/LConn3 -- T_92419253_400000_Macclesfield_Substation/RConn3 -- bus366/LConn1
  T_95338682_400000;132000_Legacy_Substation/RConn1 -- L_95338682/LConn1
  T_95338682_400000;132000_Legacy_Substation/RConn2 -- L_95338682/LConn2
  L_95338682/LConn3 -- T_95338682_400000;132000_Legacy_Substation/RConn3 -- bus367/LConn1
  T_127184694_400000;132000_/RConn1 -- L_127184694/LConn1
  T_127184694_400000;132000_/RConn2 -- L_127184694/LConn2
  L_127184694/LConn3 -- T_127184694_400000;132000_/RConn3 -- bus368/LConn1
  T_89573357_400000;275000_Trawsfynydd_Substation/RConn1 -- L_89573357/LConn1
  T_89573357_400000;275000_Trawsfynydd_Substation/RConn2 -- L_89573357/LConn2
  L_89573357/LConn3 -- T_89573357_400000;275000_Trawsfynydd_Substation/RConn3 -- bus369/LConn1
  T_193460855_400000_/RConn1 -- L_193460855/LConn1
  T_193460855_400000_/RConn2 -- L_193460855/LConn2
  L_193460855/LConn3 -- T_193460855_400000_/RConn3 -- bus370/LConn1
  T_89038614_400000;132000_Eaton_Socon_substation/RConn1 -- L_89038614/LConn1
  T_89038614_400000;132000_Eaton_Socon_substation/RConn2 -- L_89038614/LConn2
  L_89038614/LConn3 -- T_89038614_400000;132000_Eaton_Socon_substation/RConn3 -- bus371/LConn1
  T_4715504_400000;132000_Botley_Wood/RConn1 -- L_4715504/LConn1
  T_4715504_400000;132000_Botley_Wood/RConn2 -- L_4715504/LConn2
  L_4715504/LConn3 -- T_4715504_400000;132000_Botley_Wood/RConn3 -- bus372/LConn1
  T_71118628_400000_/RConn1 -- L_71118628/LConn1
  T_71118628_400000_/RConn2 -- L_71118628/LConn2
  L_71118628/LConn3 -- T_71118628_400000_/RConn3 -- bus373/LConn1
  T_103829261__/RConn1 -- L_103829261/LConn1
  T_103829261__/RConn2 -- L_103829261/LConn2
  L_103829261/LConn3 -- T_103829261__/RConn3 -- bus374/LConn1
  T_137212453__/RConn1 -- L_137212453/LConn1
  T_137212453__/RConn2 -- L_137212453/LConn2
  L_137212453/LConn3 -- T_137212453__/RConn3 -- bus375/LConn1
  T_89573358__/RConn1 -- L_89573358/LConn1
  T_89573358__/RConn2 -- L_89573358/LConn2
  L_89573358/LConn3 -- T_89573358__/RConn3 -- bus376/LConn1
  T_142845284__/RConn1 -- L_142845284/LConn1
  T_142845284__/RConn2 -- L_142845284/LConn2
  L_142845284/LConn3 -- T_142845284__/RConn3 -- bus377/LConn1
  T_23232738_400000;275000_Iver_Substation/RConn1 -- L_23232738/LConn1
  T_23232738_400000;275000_Iver_Substation/RConn2 -- L_23232738/LConn2
  L_23232738/LConn3 -- T_23232738_400000;275000_Iver_Substation/RConn3 -- bus378/LConn1
  T_41710456_400000;132000_Mop_End_Substation/RConn1 -- L_41710456/LConn1
  T_41710456_400000;132000_Mop_End_Substation/RConn2 -- L_41710456/LConn2
  L_41710456/LConn3 -- T_41710456_400000;132000_Mop_End_Substation/RConn3 -- bus379/LConn1
  T_23164132_400000;275000;132000_/RConn1 -- L_23164132/LConn1
  T_23164132_400000;275000;132000_/RConn2 -- L_23164132/LConn2
  L_23164132/LConn3 -- T_23164132_400000;275000;132000_/RConn3 -- bus380/LConn1
  T_23164256__/RConn1 -- L_23164256/LConn1
  T_23164256__/RConn2 -- L_23164256/LConn2
  L_23164256/LConn3 -- T_23164256__/RConn3 -- bus381/LConn1
  T_313495269_400000_/RConn1 -- L_313495269/LConn1
  T_313495269_400000_/RConn2 -- L_313495269/LConn2
  L_313495269/LConn3 -- T_313495269_400000_/RConn3 -- bus382/LConn1
  T_313495305__/RConn1 -- L_313495305/LConn1
  T_313495305__/RConn2 -- L_313495305/LConn2
  L_313495305/LConn3 -- T_313495305__/RConn3 -- bus383/LConn1
  T_313495302__/RConn1 -- L_313495302/LConn1
  T_313495302__/RConn2 -- L_313495302/LConn2
  L_313495302/LConn3 -- T_313495302__/RConn3 -- bus384/LConn1
  T_95279334_400000;132000_Minety/RConn1 -- L_95279334/LConn1
  T_95279334_400000;132000_Minety/RConn2 -- L_95279334/LConn2
  L_95279334/LConn3 -- T_95279334_400000;132000_Minety/RConn3 -- bus385/LConn1
  T_92460913_400000_Walham_Sub_station/RConn1 -- L_92460913/LConn1
  T_92460913_400000_Walham_Sub_station/RConn2 -- L_92460913/LConn2
  L_92460913/LConn3 -- T_92460913_400000_Walham_Sub_station/RConn3 -- bus386/LConn1
  T_96107758_400000;275000_Feckenham/RConn1 -- L_96107758/LConn1
  T_96107758_400000;275000_Feckenham/RConn2 -- L_96107758/LConn2
  L_96107758/LConn3 -- T_96107758_400000;275000_Feckenham/RConn3 -- bus387/LConn1
  T_200511209_400000;275000_Hawthorn_Pit_Substation/RConn1 -- L_200511209/LConn1
  T_200511209_400000;275000_Hawthorn_Pit_Substation/RConn2 -- L_200511209/LConn2
  L_200511209/LConn3 -- T_200511209_400000;275000_Hawthorn_Pit_Substation/RConn3 -- bus388/LConn1
  T_142397822__/RConn1 -- L_142397822/LConn1
  T_142397822__/RConn2 -- L_142397822/LConn2
  L_142397822/LConn3 -- T_142397822__/RConn3 -- bus389/LConn1
  T_109730296_400000;275000_Lackenby_Substation/RConn1 -- L_109730296/LConn1
  T_109730296_400000;275000_Lackenby_Substation/RConn2 -- L_109730296/LConn2
  L_109730296/LConn3 -- T_109730296_400000;275000_Lackenby_Substation/RConn3 -- bus390/LConn1
  T_16582436_400000;132000_Northfleet_East_Substation/RConn1 -- L_16582436/LConn1
  T_16582436_400000;132000_Northfleet_East_Substation/RConn2 -- L_16582436/LConn2
  L_16582436/LConn3 -- T_16582436_400000;132000_Northfleet_East_Substation/RConn3 -- bus391/LConn1
  T_26938722_400000;132000_Abham_Substation/RConn1 -- L_26938722/LConn1
  T_26938722_400000;132000_Abham_Substation/RConn2 -- L_26938722/LConn2
  L_26938722/LConn3 -- T_26938722_400000;132000_Abham_Substation/RConn3 -- bus392/LConn1
  T_88455233__Kingsnorth_Substation/RConn1 -- L_88455233/LConn1
  T_88455233__Kingsnorth_Substation/RConn2 -- L_88455233/LConn2
  L_88455233/LConn3 -- T_88455233__Kingsnorth_Substation/RConn3 -- bus393/LConn1
  T_308653840__/RConn1 -- L_308653840/LConn1
  T_308653840__/RConn2 -- L_308653840/LConn2
  L_308653840/LConn3 -- T_308653840__/RConn3 -- bus394/LConn1
  T_365868376_400000_New_Connahs_Quay_Substation/RConn1 -- L_365868376/LConn1
  T_365868376_400000_New_Connahs_Quay_Substation/RConn2 -- L_365868376/LConn2
  L_365868376/LConn3 -- T_365868376_400000_New_Connahs_Quay_Substation/RConn3 -- bus395/LConn1
  T_92340133_400000;132000_East_Claydon_Substation/RConn1 -- L_92340133/LConn1
  T_92340133_400000;132000_East_Claydon_Substation/RConn2 -- L_92340133/LConn2
  L_92340133/LConn3 -- T_92340133_400000;132000_East_Claydon_Substation/RConn3 -- bus396/LConn1
  T_190511290_400000;132000_/RConn1 -- L_190511290/LConn1
  T_190511290_400000;132000_/RConn2 -- L_190511290/LConn2
  L_190511290/LConn3 -- T_190511290_400000;132000_/RConn3 -- bus397/LConn1
  T_91010711_400000;25000_Singlewell_Feeder_Station/RConn1 -- L_91010711/LConn1
  T_91010711_400000;25000_Singlewell_Feeder_Station/RConn2 -- L_91010711/LConn2
  L_91010711/LConn3 -- T_91010711_400000;25000_Singlewell_Feeder_Station/RConn3 -- bus398/LConn1
  T_292470577_400000_Electric_Sub_Station/RConn1 -- L_292470577/LConn1
  T_292470577_400000_Electric_Sub_Station/RConn2 -- L_292470577/LConn2
  L_292470577/LConn3 -- T_292470577_400000_Electric_Sub_Station/RConn3 -- bus399/LConn1
  T_142843255__/RConn1 -- L_142843255/LConn1
  T_142843255__/RConn2 -- L_142843255/LConn2
  L_142843255/LConn3 -- T_142843255__/RConn3 -- bus400/LConn1
  T_280317944__St_Asaph_Substation/RConn1 -- L_280317944/LConn1
  T_280317944__St_Asaph_Substation/RConn2 -- L_280317944/LConn2
  L_280317944/LConn3 -- T_280317944__St_Asaph_Substation/RConn3 -- bus401/LConn1
  T_290606955__/RConn1 -- L_290606955/LConn1
  T_290606955__/RConn2 -- L_290606955/LConn2
  L_290606955/LConn3 -- T_290606955__/RConn3 -- bus402/LConn1
  T_193460868__/RConn1 -- L_193460868/LConn1
  T_193460868__/RConn2 -- L_193460868/LConn2
  L_193460868/LConn3 -- T_193460868__/RConn3 -- bus403/LConn1
  T_313180501_400000_/RConn1 -- L_313180501/LConn1
  T_313180501_400000_/RConn2 -- L_313180501/LConn2
  L_313180501/LConn3 -- T_313180501_400000_/RConn3 -- bus404/LConn1
  T_310488541__/RConn1 -- L_310488541/LConn1
  T_310488541__/RConn2 -- L_310488541/LConn2
  L_310488541/LConn3 -- T_310488541__/RConn3 -- bus405/LConn1
  T_263863442__Didcot_Substation/RConn1 -- L_263863442/LConn1
  T_263863442__Didcot_Substation/RConn2 -- L_263863442/LConn2
  L_263863442/LConn3 -- T_263863442__Didcot_Substation/RConn3 -- bus406/LConn1
  T_92483460__/RConn1 -- L_92483460/LConn1
  T_92483460__/RConn2 -- L_92483460/LConn2
  L_92483460/LConn3 -- T_92483460__/RConn3 -- bus407/LConn1
  T_88287125_400000;132000_/RConn1 -- L_88287125/LConn1
  T_88287125_400000;132000_/RConn2 -- L_88287125/LConn2
  L_88287125/LConn3 -- T_88287125_400000;132000_/RConn3 -- bus408/LConn1
  T_90534270_400000;132000_/RConn1 -- L_90534270/LConn1
  T_90534270_400000;132000_/RConn2 -- L_90534270/LConn2
  L_90534270/LConn3 -- T_90534270_400000;132000_/RConn3 -- bus409/LConn1
  T_31015820_400000;132000;66000_St_John's_Wood_substation/RConn1 -- L_31015820/LConn1
  T_31015820_400000;132000;66000_St_John's_Wood_substation/RConn2 -- L_31015820/LConn2
  L_31015820/LConn3 -- T_31015820_400000;132000;66000_St_John's_Wood_substation/RConn3 -- bus410/LConn1
  T_371757485_400000;275000_/RConn1 -- L_371757485/LConn1
  T_371757485_400000;275000_/RConn2 -- L_371757485/LConn2
  L_371757485/LConn3 -- T_371757485_400000;275000_/RConn3 -- bus411/LConn1
  T_315965849__/RConn1 -- L_315965849/LConn1
  T_315965849__/RConn2 -- L_315965849/LConn2
  L_315965849/LConn3 -- T_315965849__/RConn3 -- bus412/LConn1
  T_264102298_400000;275000_/RConn1 -- L_264102298/LConn1
  T_264102298_400000;275000_/RConn2 -- L_264102298/LConn2
  L_264102298/LConn3 -- T_264102298_400000;275000_/RConn3 -- bus413/LConn1
  T_160173034__/RConn1 -- L_160173034/LConn1
  T_160173034__/RConn2 -- L_160173034/LConn2
  L_160173034/LConn3 -- T_160173034__/RConn3 -- bus414/LConn1
  T_23167419_400000_/RConn1 -- L_23167419/LConn1
  T_23167419_400000_/RConn2 -- L_23167419/LConn2
  L_23167419/LConn3 -- T_23167419_400000_/RConn3 -- bus415/LConn1
  T_160580052_400000_/RConn1 -- L_160580052/LConn1
  T_160580052_400000_/RConn2 -- L_160580052/LConn2
  L_160580052/LConn3 -- T_160580052_400000_/RConn3 -- bus416/LConn1
  T_292471784_400000;132000_/RConn1 -- L_292471784/LConn1
  T_292471784_400000;132000_/RConn2 -- L_292471784/LConn2
  L_292471784/LConn3 -- T_292471784_400000;132000_/RConn3 -- bus417/LConn1
  T_160173033__/RConn1 -- L_160173033/LConn1
  T_160173033__/RConn2 -- L_160173033/LConn2
  L_160173033/LConn3 -- T_160173033__/RConn3 -- bus418/LConn1
  T_314338799_400000_/RConn1 -- L_314338799/LConn1
  T_314338799_400000_/RConn2 -- L_314338799/LConn2
  L_314338799/LConn3 -- T_314338799_400000_/RConn3 -- bus419/LConn1
